simulink model "ABB_1010"  (R2024a)
settings: Solver=VariableStepAuto  StartTime=0.0  StopTime=200  RelTol=1e-3
model workspace: external: MATLAB File C:\Users\lucas\OneDrive\Documents\MATLAB\projeto final\ABB_1010_DataFile.m (data not in the file)
values from neighbouring files (symbols this model uses):
  g = 9.81    [inicializacaoAntropomorfico.m]
  I1 = [ 0.00243841  0.00000307  0.00007261    [inicializacaoAntropomorfico.m]
  I2 = [ 0.01633569  0.00000387 -0.00034405    [inicializacaoAntropomorfico.m]
  I3 = [ 0.00244760 -0.00000208  0.00000538    [inicializacaoAntropomorfico.m]
  I4 = [ 0.00245792 -0.00000008  0.00003121    [inicializacaoAntropomorfico.m]
  I5 = [ 0.00062165 -0.00000206 -0.00000303    [inicializacaoAntropomorfico.m]
  I6 = [ 0.00000357  0.00000000  0.00000000    [inicializacaoAntropomorfico.m]
  I7 = [(m7*L7^2)/12 0.00000000  0.00000000    [inicializacaoAntropomorfico.m]
  L = [L1, L2, L3, L4, L5, L6, L7]    [inicializacaoAntropomorfico.m]
  Lcm1 = [-0.00258308  0.00024508 -0.01434968]    [inicializacaoAntropomorfico.m]
  Lcm2 = [-0.02078894  0.00020016 -0.10516734]    [inicializacaoAntropomorfico.m]
  Lcm3 = [ 0.00021912  0.00015355 -0.06228290]    [inicializacaoAntropomorfico.m]
  Lcm4 = [-0.00172658 -0.00124140 -0.07369196]    [inicializacaoAntropomorfico.m]
  Lcm5 = [-0.00014110  0.00085992 -0.03825278]    [inicializacaoAntropomorfico.m]
  Lcm6 = [ 0.00002478  0.00000000 -0.00042157]    [inicializacaoAntropomorfico.m]
  Lcm7 = [ 0           0          -0.05000000]    [inicializacaoAntropomorfico.m]
  m = [m1, m2, m3, m4, m5, m6, m7]    [inicializacaoAntropomorfico.m]
  Pf = [  0.05    [inicializacaoAntropomorfico.m]
  Pi = [  0.2    [inicializacaoAntropomorfico.m]
  Raio = [0]    [inicializacaoAntropomorfico.m]
  Sentido = [0]    [inicializacaoAntropomorfico.m]
  Tipo = [1]    [inicializacaoAntropomorfico.m]
undefined symbols (not defined in the file or in its folder): smiData, X, Y, Z
libraries: sm_lib x35, nesl_utility x7
(part 2 of 16)

== matlab function ABB_1010/Dinamica1/MATLAB Function ==
  data: M output; I1 parameter; L parameter; Lcm1 parameter; Q input; I2 parameter; I3 parameter; I4 parameter; I5 parameter; I6 parameter; Lcm2 parameter; Lcm3 parameter; Lcm4 parameter; Lcm5 parameter; Lcm6 parameter; m parameter; Lcm7 parameter; I7 parameter
function M = func_M(I1, L, Lcm1, Q, I2, I3, I4, I5, I6, Lcm2, Lcm3, Lcm4, Lcm5, Lcm6, m, Lcm7, I7)
%func_M
%    OUT1 = func_M(Ixx2,Ixx3,Ixx4,Ixx5,Ixx6,Ixy2,Ixy3,Ixy4,Ixy5,Ixy6,Ixz2,Ixz3,Ixz4,Ixz5,Ixz6,Iyx2,Iyx3,Iyx4,Iyx5,Iyx6,Iyy2,Iyy3,Iyy4,Iyy5,Iyy6,Iyz2,Iyz3,Iyz4,Iyz5,Iyz6,Izx2,Izx3,Izx4,Izx5,Izx6,Izy2,Izy3,Izy4,Izy5,Izy6,Izz1,Izz2,Izz3,Izz4,Izz5,Izz6,Lx2,Lx3,Lxcm1,Lxcm2,Lxcm3,Lxcm4,Lxcm5,Lxcm6,Lycm1,Lycm2,Lycm3,Lycm4,Lycm5,Lycm6,Lz4,Lz5,Lzcm2,Lzcm3,Lzcm4,Lzcm5,Lzcm6,Q1,Q2,Q3,Q4,Q5,Q6,M1,M2,M3,M4,M5,M6)
    
%    This function was generated by the Symbolic Math Toolbox version 24.1.
%    30-Apr-2025 07:30:44

M = zeros(6,6);

m1  = m(1);
m2  = m(2);
m3  = m(3);
m4  = m(4);
m5  = m(5);
m6  = m(6);
m7  = m(7);

Q1  = Q(1);
Q2  = Q(2);
Q3  = Q(3);
Q4  = Q(4);
Q5  = Q(5);
Q6  = Q(6);

Lz1 = L(1);
Lx2 = L(2);
Lx3 = L(3);
Lx4 = L(4);
Lz5 = L(5);
Lz6 = L(6);
Lz7 = L(7);

Lxcm1 = Lcm1(1);
Lycm1 = Lcm1(2);
Lzcm1 = Lcm1(3);

Lxcm2 = Lcm2(1);
Lycm2 = Lcm2(2);
Lzcm2 = Lcm2(3);

Lxcm3 = Lcm3(1);
Lycm3 = Lcm3(2);
Lzcm3 = Lcm3(3);

Lxcm4 = Lcm4(1);
Lycm4 = Lcm4(2);
Lzcm4 = Lcm4(3);

Lxcm5 = Lcm5(1);
Lycm5 = Lcm5(2);
Lzcm5 = Lcm5(3);

Lxcm6 = Lcm6(1);
Lycm6 = Lcm6(2);
Lzcm6 = Lcm6(3);

Lxcm7 = Lcm7(1);
Lycm7 = Lcm7(2);
Lzcm7 = Lcm7(3);

Ixx1 = I1(1,1);
Ixy1 = I1(1,2);
Ixz1 = I1(1,3);
Iyx1 = I1(2,1);
Iyy1 = I1(2,2);
Iyz1 = I1(2,3);
Izx1 = I1(3,1);
Izy1 = I1(3,2);
Izz1 = I1(3,3);

Ixx2 = I2(1,1);
Ixy2 = I2(1,2);
Ixz2 = I2(1,3);
Iyx2 = I2(2,1);
Iyy2 = I2(2,2);
Iyz2 = I2(2,3);
Izx2 = I2(3,1);
Izy2 = I2(3,2);
Izz2 = I2(3,3);

Ixx3 = I3(1,1);
Ixy3 = I3(1,2);
Ixz3 = I3(1,3);
Iyx3 = I3(2,1);
Iyy3 = I3(2,2);
Iyz3 = I3(2,3);
Izx3 = I3(3,1);
Izy3 = I3(3,2);
Izz3 = I3(3,3);

Ixx4 = I4(1,1);
Ixy4 = I4(1,2);
Ixz4 = I4(1,3);
Iyx4 = I4(2,1);
Iyy4 = I4(2,2);
Iyz4 = I4(2,3);
Izx4 = I4(3,1);
Izy4 = I4(3,2);
Izz4 = I4(3,3);

Ixx5 = I5(1,1);
Ixy5 = I5(1,2);
Ixz5 = I5(1,3);
Iyx5 = I5(2,1);
Iyy5 = I5(2,2);
Iyz5 = I5(2,3);
Izx5 = I5(3,1);
Izy5 = I5(3,2);
Izz5 = I5(3,3);

Ixx6 = I6(1,1);
Ixy6 = I6(1,2);
Ixz6 = I6(1,3);
Iyx6 = I6(2,1);
Iyy6 = I6(2,2);
Iyz6 = I6(2,3);
Izx6 = I6(3,1);
Izy6 = I6(3,2);
Izz6 = I6(3,3);

Ixx7 = I7(1,1);
Ixy7 = I7(1,2);
Ixz7 = I7(1,3);
Iyx7 = I7(2,1);
Iyy7 = I7(2,2);
Iyz7 = I7(2,3);
Izx7 = I7(3,1);
Izy7 = I7(3,2);
Izz7 = I7(3,3);

t2 = cos(Q1);
t3 = cos(Q2);
t4 = cos(Q3);
t5 = cos(Q4);
t6 = cos(Q5);
t7 = cos(Q6);
t8 = sin(Q1);
t9 = sin(Q2);
t10 = sin(Q3);
t11 = sin(Q4);
t12 = sin(Q5);
t13 = sin(Q6);
t14 = Q2+Q3;
t15 = Lx2^2;
t16 = Lx3^2;
t17 = Lx4^2;
t18 = Lxcm3^2;
t19 = Lxcm4^2;
t20 = Lxcm5^2;
t21 = Lxcm6^2;
t22 = Lycm4^2;
t23 = Lycm5^2;
t24 = Lycm6^2;
t25 = Lz6^2;
t26 = Lzcm3^2;
t27 = Lzcm4^2;
t28 = Lzcm5^2;
t29 = Lzcm6^2;
t30 = Q4*2.0;
t31 = Q5*2.0;
t32 = Q6*2.0;
t33 = Lz6+Lzcm6;
t50 = Lx3*Lxcm3*m3*2.0;
t51 = Lz6*Lzcm6*m6*2.0;
t34 = t5^2;
t35 = t6^2;
t36 = t7^2;
t37 = sin(t30);
t38 = sin(t31);
t39 = sin(t32);
t40 = t11^2;
t41 = t12^2;
t42 = t13^2;
t43 = Ixx6*t5;
t44 = Iyy5*t5;
t45 = Izz6*t6;
t46 = Lycm6*t7;
t47 = cos(t14);
t48 = Lxcm6*t13;
t49 = sin(t14);
t52 = m3*t16;
t53 = m4*t16;
t54 = m5*t16;
t55 = m6*t16;
t56 = m3*t18;
t57 = m5*t20;
t58 = m6*t21;
t59 = m4*t22;
t60 = m5*t23;
t61 = m6*t24;
t62 = m6*t25;
t63 = m3*t26;
t64 = m4*t27;
t65 = m5*t28;
t66 = m6*t29;
t67 = t2*t5;
t68 = t2*t11;
t69 = t5*t8;
t70 = t8*t11;
t71 = Ixx5*t3*t4;
t72 = Iyy6*t3*t4;
t73 = Izz4*t3*t4;
t74 = Lx2*t2*t3;
t75 = Lx2*Lx3*m3*t4;
t76 = Lx2*Lx3*m4*t4;
t77 = Lx2*Lx3*m5*t4;
t78 = Lx2*Lx3*m6*t4;
t79 = Lx2*Lxcm3*m3*t4;
t80 = Lx3*Lxcm5*m5*t6;
t81 = Lx4*Lxcm6*m6*t7;
t82 = Lycm2*Lzcm2*m2*t3;
t83 = Lycm4*Lzcm4*m4*t5;
t84 = Lycm5*Lzcm5*m5*t6;
t85 = Lx2*t3*t8;
t86 = Lx2*Lycm2*m2*t9;
t87 = Lx2*Lycm3*m3*t9;
t88 = Lx4*Lycm6*m6*t13;
t89 = Lxcm2*Lycm2*m2*t9;
t90 = Lxcm5*Lycm5*m5*t12;
t91 = Lxcm6*Lycm6*m6*t12;
t92 = Lx3*Lz6*m6*t12;
t93 = Lx2*Lzcm3*m3*t10;
t94 = Lx2*Lzcm4*m4*t10;
t95 = Lx4*Lzcm4*m4*t11;
t96 = Lx3*Lzcm5*m5*t12;
t97 = Lx3*Lzcm6*m6*t12;
t98 = Lxcm4*Lzcm4*m4*t11;
t99 = Lxcm5*Lzcm5*m5*t11;
t100 = Ixx5*t9*t10;
t101 = Iyy6*t9*t10;
t102 = Izz4*t9*t10;
t103 = Izz6*t11*t12;
t118 = Lx3*Lx4*m4*t5*2.0;
t119 = Lx3*Lx4*m5*t5*2.0;
t120 = Lx3*Lx4*m6*t5*2.0;
t121 = Lx3*Lxcm4*m4*t5*2.0;
t122 = t5*t51;
t123 = Lx3*Lycm4*m4*t11*2.0;
t124 = Lx3*Lycm5*m5*t11*2.0;
t133 = t2*t3*t4;
t135 = t2*t3*t10;
t136 = t2*t4*t9;
t137 = t3*t4*t8;
t138 = t2*t9*t10;
t139 = t3*t8*t10;
t140 = t4*t8*t9;
t141 = t8*t9*t10;
t170 = Lx2*Lx4*m4*t3*t5;
t171 = Lx2*Lx4*m4*t4*t5;
t172 = Lx2*Lx4*m5*t3*t5;
t173 = Lx2*Lx4*m5*t4*t5;
t174 = Lx2*Lx4*m6*t3*t5;
t175 = Lx2*Lx4*m6*t4*t5;
t176 = Lx2*Lxcm4*m4*t3*t5;
t177 = Lx2*Lxcm4*m4*t4*t5;
t178 = Lx2*Lxcm5*m5*t4*t6;
t179 = Lx4*Lxcm5*m5*t5*t6;
t180 = Lx3*Lxcm6*m6*t6*t7;
t183 = Lycm3*Lzcm3*m3*t3*t4;
t189 = Lx3*Lycm3*m3*t3*t10;
t190 = Lx3*Lycm3*m3*t4*t9;
t191 = Lx2*Lycm4*m4*t3*t11;
t192 = Lx2*Lycm4*m4*t5*t9;
t193 = Lx2*Lycm4*m4*t4*t11;
t194 = Lx2*Lycm4*m4*t5*t10;
t195 = Lx4*Lycm4*m4*t3*t10;
t196 = Lx4*Lycm4*m4*t4*t9;
t197 = Lx2*Lycm5*m5*t3*t11;
t198 = Lx2*Lycm5*m5*t5*t9;
t199 = Lx2*Lycm5*m5*t4*t11;
t200 = Lx2*Lycm5*m5*t5*t10;
t201 = Lx4*Lycm5*m5*t3*t10;
t202 = Lx4*Lycm5*m5*t4*t9;
t203 = Lx3*Lycm6*m6*t6*t13;
t205 = Lxcm3*Lycm3*m3*t3*t10;
t206 = Lxcm3*Lycm3*m3*t4*t9;
t207 = Lxcm4*Lycm4*m4*t3*t10;
t208 = Lxcm4*Lycm4*m4*t4*t9;
t210 = Lxcm5*Lycm5*m5*t6*t11;
t212 = Lxcm6*Lycm6*m6*t6*t11;
t213 = Lx2*Lz6*m6*t4*t12;
t214 = Lx2*Lz6*m6*t6*t10;
t215 = Lx4*Lz6*m6*t5*t12;
t216 = Lx4*Lz6*m6*t6*t11;
t217 = Lx2*Lzcm5*m5*t4*t12;
t218 = Lx2*Lzcm5*m5*t6*t10;
t219 = Lx2*Lzcm6*m6*t4*t12;
t220 = Lx2*Lzcm6*m6*t6*t10;
t221 = Lx4*Lzcm5*m5*t5*t12;
t222 = Lx4*Lzcm5*m5*t6*t11;
t223 = Lx4*Lzcm6*m6*t5*t12;
t224 = Lx4*Lzcm6*m6*t6*t11;
t226 = Lxcm6*Lz6*m6*t7*t11;
t228 = Lxcm6*Lz6*m6*t7*t12;
t230 = Lxcm6*Lzcm6*m6*t7*t11;
t232 = Lxcm6*Lzcm6*m6*t7*t12;
t233 = Ixx6*t3*t10*t11;
t234 = Ixx6*t4*t9*t11;
t235 = Ixx5*t6*t11*t12;
t236 = Ixx6*t7*t12*t13;
t237 = Iyy5*t3*t10*t11;
t238 = Iyy5*t4*t9*t11;
t239 = Iyy6*t6*t11*t12;
t240 = Iyy6*t7*t12*t13;
t242 = Izz5*t6*t11*t12;
t244 = Lx2*Lx4*m4*t9*t11;
t245 = Lx2*Lx4*m4*t10*t11;
t246 = Lx2*Lx4*m5*t9*t11;
t247 = Lx2*Lx4*m5*t10*t11;
t248 = Lx2*Lx4*m6*t9*t11;
t249 = Lx2*Lx4*m6*t10*t11;
t250 = Lx2*Lxcm4*m4*t9*t11;
t251 = Lx2*Lxcm4*m4*t10*t11;
t252 = Lx2*Lxcm5*m5*t10*t12;
t253 = Lx4*Lxcm5*m5*t11*t12;
t255 = Lycm6*Lz6*m6*t11*t13;
t256 = Lycm6*Lz6*m6*t12*t13;
t257 = Lycm3*Lzcm3*m3*t9*t10;
t258 = Lycm5*Lzcm5*m5*t11*t12;
t259 = Lycm6*Lzcm6*m6*t11*t13;
t260 = Lycm6*Lzcm6*m6*t12*t13;
t261 = m4*t9*t10*t17;
t262 = m5*t9*t10*t17;
t263 = m6*t9*t10*t17;
t264 = m4*t9*t10*t19;
t298 = Lx4*Lxcm4*m4*t3*t4*2.0;
t300 = t3*t4*t51;
t305 = m4*t3*t4*t17;
t306 = m5*t3*t4*t17;
t307 = m6*t3*t4*t17;
t308 = m4*t3*t4*t19;
t315 = Lx4*Lxcm4*m4*t9*t10*2.0;
t317 = t9*t10*t51;
t331 = Lx3*Lx4*m4*t3*t4*t5;
t332 = Lx3*Lx4*m5*t3*t4*t5;
t333 = Lx3*Lx4*m6*t3*t4*t5;
t334 = Lx3*Lxcm4*m4*t3*t4*t5;
t335 = Lx2*Lxcm5*m5*t3*t5*t6;
t337 = Lx2*Lxcm6*m6*t3*t5*t7;
t339 = Lx2*Lxcm6*m6*t4*t6*t7;
t350 = Lx3*Lycm4*m4*t3*t4*t11;
t351 = Lx3*Lycm4*m4*t3*t5*t10;
t352 = Lx3*Lycm4*m4*t4*t5*t9;
t353 = Lx3*Lycm5*m5*t3*t4*t11;
t354 = Lx3*Lycm5*m5*t3*t5*t10;
t355 = Lx3*Lycm5*m5*t4*t5*t9;
t356 = Lx2*Lycm6*m6*t3*t5*t13;
t364 = Lx2*Lycm6*m6*t4*t6*t13;
t369 = Lxcm5*Lycm5*m5*t3*t6*t10;
t370 = Lxcm5*Lycm5*m5*t4*t6*t9;
t372 = Lxcm6*Lycm6*m6*t3*t6*t10;
t373 = Lxcm6*Lycm6*m6*t4*t6*t9;
t374 = Lx2*Lz6*m6*t3*t5*t12;
t375 = Lx2*Lz6*m6*t3*t6*t11;
t379 = Lx4*Lzcm4*m4*t3*t5*t10;
t380 = Lx4*Lzcm4*m4*t4*t5*t9;
t381 = Lx2*Lzcm5*m5*t3*t5*t12;
t382 = Lx2*Lzcm5*m5*t3*t6*t11;
t385 = Lx2*Lzcm6*m6*t3*t5*t12;
t386 = Lx2*Lzcm6*m6*t3*t6*t11;
t392 = Lxcm4*Lzcm4*m4*t3*t5*t10;
t393 = Lxcm4*Lzcm4*m4*t4*t5*t9;
t395 = Lxcm5*Lzcm5*m5*t3*t5*t10;
t396 = Lxcm5*Lzcm5*m5*t4*t5*t9;
t402 = Ixx4*t3*t5*t10*t11;
t403 = Ixx4*t4*t5*t9*t11;
t407 = Ixx6*t6*t7*t11*t13;
t408 = Iyy4*t3*t5*t10*t11;
t409 = Iyy4*t4*t5*t9*t11;
t413 = Iyy6*t6*t7*t11*t13;
t414 = Izz5*t3*t5*t10*t11;
t415 = Izz5*t4*t5*t9*t11;
t416 = Izz6*t3*t5*t10*t11;
t417 = Izz6*t4*t5*t9*t11;
t418 = Izz6*t3*t5*t10*t12;
t419 = Izz6*t4*t5*t9*t12;
t422 = Lx3*Lx4*m4*t3*t10*t11;
t423 = Lx3*Lx4*m4*t4*t9*t11;
t424 = Lx3*Lx4*m4*t5*t9*t10;
t425 = Lx3*Lx4*m5*t3*t10*t11;
t426 = Lx3*Lx4*m5*t4*t9*t11;
t427 = Lx3*Lx4*m5*t5*t9*t10;
t428 = Lx3*Lx4*m6*t3*t10*t11;
t429 = Lx3*Lx4*m6*t4*t9*t11;
t430 = Lx3*Lx4*m6*t5*t9*t10;
t431 = Lx3*Lxcm4*m4*t3*t10*t11;
t432 = Lx3*Lxcm4*m4*t4*t9*t11;
t433 = Lx3*Lxcm4*m4*t5*t9*t10;
t434 = Lx2*Lxcm5*m5*t3*t11*t12;
t435 = Lx2*Lxcm5*m5*t6*t9*t11;
t437 = Lx2*Lxcm5*m5*t6*t10*t11;
t442 = Lx2*Lxcm6*m6*t7*t10*t11;
t447 = Lx2*Lxcm6*m6*t7*t10*t12;
t452 = Lycm4*Lzcm4*m4*t3*t10*t11;
t453 = Lycm4*Lzcm4*m4*t4*t9*t11;
t455 = Lycm5*Lzcm5*m5*t3*t10*t12;
t456 = Lycm5*Lzcm5*m5*t4*t9*t12;
t460 = Lx3*Lycm4*m4*t9*t10*t11;
t461 = Lx3*Lycm5*m5*t9*t10*t11;
t462 = Lx2*Lycm6*m6*t10*t11*t13;
t464 = Lx2*Lycm6*m6*t10*t12*t13;
t468 = Lx2*Lz6*m6*t9*t11*t12;
t469 = Lx2*Lz6*m6*t10*t11*t12;
t471 = Lx2*Lzcm5*m5*t9*t11*t12;
t472 = Lx2*Lzcm5*m5*t10*t11*t12;
t473 = Lx2*Lzcm6*m6*t9*t11*t12;
t474 = Lx2*Lzcm6*m6*t10*t11*t12;
t535 = Lz6*Lzcm6*m6*t9*t10*-2.0;
t555 = Lx4*Lxcm5*m5*t3*t4*t6*2.0;
t567 = Lx4*Lz6*m6*t3*t4*t12*2.0;
t568 = Lx4*Lzcm5*m5*t3*t4*t12*2.0;
t569 = Lx4*Lzcm6*m6*t3*t4*t12*2.0;
t574 = Lx4*Lxcm5*m5*t6*t9*t10*2.0;
t579 = t3*t10*t11*t51;
t580 = t4*t9*t11*t51;
t582 = Lx4*Lz6*m6*t9*t10*t12*2.0;
t583 = Lx4*Lzcm5*m5*t9*t10*t12*2.0;
t584 = Lx4*Lzcm6*m6*t9*t10*t12*2.0;
t613 = Lx3*Lxcm6*m6*t3*t4*t5*t7;
t628 = Lx3*Lycm6*m6*t3*t4*t5*t13;
t643 = Lx3*Lz6*m6*t3*t4*t6*t11;
t645 = Lx4*Lz6*m6*t3*t5*t6*t10;
t646 = Lx4*Lz6*m6*t4*t5*t6*t9;
t648 = Lx3*Lzcm5*m5*t3*t4*t6*t11;
t650 = Lx4*Lzcm5*m5*t3*t5*t6*t10;
t651 = Lx4*Lzcm5*m5*t4*t5*t6*t9;
t653 = Lx3*Lzcm6*m6*t3*t4*t6*t11;
t655 = Lx4*Lzcm6*m6*t3*t5*t6*t10;
t656 = Lx4*Lzcm6*m6*t4*t5*t6*t9;
t658 = Lxcm6*Lz6*m6*t3*t5*t7*t10;
t659 = Lxcm6*Lz6*m6*t4*t5*t7*t9;
t663 = Lxcm6*Lzcm6*m6*t3*t5*t7*t10;
t664 = Lxcm6*Lzcm6*m6*t4*t5*t7*t9;
t671 = Ixx5*t3*t5*t6*t10*t12;
t672 = Ixx5*t4*t5*t6*t9*t12;
t674 = Ixx6*t3*t6*t7*t10*t13;
t675 = Ixx6*t4*t6*t7*t9*t13;
t677 = Iyy6*t3*t5*t6*t10*t12;
t678 = Iyy6*t4*t5*t6*t9*t12;
t680 = Iyy6*t3*t6*t7*t10*t13;
t681 = Iyy6*t4*t6*t7*t9*t13;
t683 = Izz5*t3*t5*t6*t10*t12;
t684 = Izz5*t4*t5*t6*t9*t12;
t691 = Lx3*Lxcm5*m5*t3*t4*t11*t12;
t696 = Lx4*Lxcm5*m5*t3*t5*t10*t12;
t697 = Lx4*Lxcm5*m5*t3*t6*t10*t11;
t698 = Lx4*Lxcm5*m5*t4*t5*t9*t12;
t699 = Lx4*Lxcm5*m5*t4*t6*t9*t11;
t703 = Lx3*Lxcm6*m6*t5*t7*t9*t10;
t705 = Lx2*Lxcm6*m6*t3*t7*t11*t12;
t706 = Lx2*Lxcm6*m6*t6*t7*t9*t11;
t711 = Lycm6*Lz6*m6*t3*t5*t10*t13;
t713 = Lycm6*Lz6*m6*t4*t5*t9*t13;
t725 = Lycm6*Lzcm6*m6*t3*t5*t10*t13;
t727 = Lycm6*Lzcm6*m6*t4*t5*t9*t13;
t736 = Lx3*Lycm6*m6*t5*t9*t10*t13;
t738 = Lx2*Lycm6*m6*t3*t11*t12*t13;
t739 = Lx2*Lycm6*m6*t6*t9*t11*t13;
t751 = Lx3*Lz6*m6*t6*t9*t10*t11;
t752 = Lx4*Lz6*m6*t3*t10*t11*t12;
t753 = Lx4*Lz6*m6*t4*t9*t11*t12;
t758 = Lx3*Lzcm5*m5*t6*t9*t10*t11;
t759 = Lx4*Lzcm5*m5*t3*t10*t11*t12;
t760 = Lx4*Lzcm5*m5*t4*t9*t11*t12;
t765 = Lx3*Lzcm6*m6*t6*t9*t10*t11;
t766 = Lx4*Lzcm6*m6*t3*t10*t11*t12;
t767 = Lx4*Lzcm6*m6*t4*t9*t11*t12;
t789 = Lx3*Lxcm5*m5*t9*t10*t11*t12;
t867 = Lz6*Lzcm6*m6*t6*t11*t12*-2.0;
t909 = Lxcm5*Lzcm5*m5*t3*t4*t6*t12*2.0;
t912 = Lx4*Lxcm4*m4*t3*t5*t10*t11*2.0;
t913 = Lx4*Lxcm4*m4*t4*t5*t9*t11*2.0;
t925 = Lxcm5*Lzcm5*m5*t6*t9*t10*t12*2.0;
t927 = m4*t3*t5*t10*t11*t17;
t928 = m4*t4*t5*t9*t11*t17;
t929 = m5*t3*t5*t10*t11*t17;
t930 = m5*t4*t5*t9*t11*t17;
t931 = m6*t3*t5*t10*t11*t17;
t932 = m6*t4*t5*t9*t11*t17;
t933 = m4*t3*t5*t10*t11*t19;
t934 = m4*t4*t5*t9*t11*t19;
t1007 = Lx3*Lxcm6*m6*t3*t4*t7*t11*t12;
t1032 = Lx3*Lycm6*m6*t3*t4*t11*t12*t13;
t1061 = Lx3*Lxcm6*m6*t7*t9*t10*t11*t12;
t1071 = Lx3*Lycm6*m6*t9*t10*t11*t12*t13;
t104 = Ixx4*t34;
t105 = Ixx5*t35;
t106 = Ixx6*t34;
t107 = Ixx6*t36;
t108 = Iyy4*t34;
t109 = Iyy5*t34;
t110 = Iyy6*t35;
t111 = Iyy6*t36;
t112 = Izz5*t34;
t113 = Izz5*t35;
t114 = Izz6*t34;
t115 = Izz6*t35;
t116 = t47^2;
t117 = t49^2;
t125 = t5*t57;
t126 = t6*t58;
t127 = t5*t61;
t128 = t6*t61;
t129 = t5*t62;
t130 = t5*t65;
t131 = t5*t66;
t132 = t6*t47;
t134 = t12*t47;
t144 = -t82;
t145 = -t83;
t146 = -t84;
t147 = -t123;
t148 = -t124;
t149 = -t88;
t150 = -t91;
t151 = -t95;
t152 = -t98;
t153 = -t100;
t154 = -t101;
t155 = -t102;
t156 = t36*t43;
t158 = Lx4*Lycm4*m4*t37;
t159 = Lx4*Lycm5*m5*t37;
t160 = Lxcm4*Lycm4*m4*t37;
t161 = Lxcm6*Lycm6*m6*t39;
t162 = Lxcm5*Lzcm5*m5*t38;
t168 = t3*t4*t45;
t169 = Lycm3*Lzcm3*m3*t47;
t181 = Lz6*m6*t5*t46;
t182 = Lz6*m6*t6*t46;
t184 = t5*t84;
t185 = Lzcm6*m6*t5*t46;
t186 = Lzcm6*m6*t6*t46;
t187 = Lx3*Lycm3*m3*t49;
t188 = Lxcm3*Lycm3*m3*t49;
t204 = Lx3*m6*t12*t46;
t209 = t5*t90;
t211 = t5*t91;
t225 = Lz6*m6*t5*t48;
t227 = Lz6*m6*t6*t48;
t229 = Lzcm6*m6*t5*t48;
t231 = Lzcm6*m6*t6*t48;
t241 = t9*t10*t45;
t243 = t11*t12*t45;
t254 = Lx3*m6*t12*t48;
t265 = t9*t10*t58;
t266 = t11*t12*t58;
t267 = t9*t10*t59;
t268 = t9*t10*t60;
t269 = t11*t12*t61;
t270 = t9*t10*t62;
t271 = t9*t10*t65;
t272 = t9*t10*t66;
t273 = t46+t48;
t274 = t5*t6*t49;
t275 = t5*t12*t49;
t276 = Lx4*Lxcm4*m4*t34*2.0;
t277 = t34*t51;
t278 = t35*t51;
t279 = m4*t17*t34;
t280 = m5*t17*t34;
t281 = m6*t17*t34;
t282 = m4*t19*t34;
t283 = t35*t57;
t284 = t34*t58;
t285 = t36*t58;
t286 = t34*t59;
t287 = t34*t60;
t288 = t35*t61;
t289 = t36*t61;
t290 = t34*t62;
t291 = t35*t62;
t292 = t34*t65;
t293 = t35*t65;
t294 = t34*t66;
t295 = t35*t66;
t296 = -t138;
t297 = -t141;
t299 = t5*t80*2.0;
t301 = Lx3*m6*t11*t46*2.0;
t302 = t5*t92*2.0;
t303 = t5*t96*2.0;
t304 = t5*t97*2.0;
t309 = t3*t4*t58;
t310 = t3*t4*t59;
t311 = t3*t4*t60;
t312 = t3*t4*t62;
t313 = t3*t4*t65;
t314 = t3*t4*t66;
t316 = Lx3*m6*t11*t48*2.0;
t318 = t35*t71;
t320 = t35*t72;
t321 = t36*t72;
t324 = t35*t100;
t326 = t35*t101;
t327 = t36*t101;
t336 = t5*t178;
t338 = t3*t4*t81;
t340 = t5*t6*t81;
t349 = Lx3*Lycm5*m5*t5*t49;
t357 = Lx2*m6*t3*t11*t46;
t358 = Lx2*m6*t5*t9*t46;
t359 = Lx2*m6*t4*t11*t46;
t360 = Lx2*m6*t5*t10*t46;
t361 = t3*t4*t88;
t362 = Lx4*m6*t3*t10*t46;
t363 = Lx4*m6*t4*t9*t46;
t365 = Lx2*m6*t4*t12*t46;
t366 = t5*t6*t88;
t367 = Lx4*m6*t5*t12*t46;
t368 = t3*t4*t90;
t371 = t3*t4*t91;
t376 = t5*t213;
t377 = t5*t214;
t383 = t5*t217;
t384 = t5*t218;
t387 = t5*t219;
t388 = t5*t220;
t390 = t6*t226;
t394 = t3*t4*t99;
t398 = t6*t230;
t399 = Ixx4*t5*t11*t49;
t400 = Iyy4*t5*t11*t49;
t401 = t11*t44*t49;
t404 = t3*t10*t11*t43;
t405 = t4*t9*t11*t43;
t406 = t7*t12*t13*t43;
t410 = t3*t10*t11*t44;
t411 = t4*t9*t11*t44;
t412 = t5*t240;
out1 = ft_1({Ixx2,Ixx3,Ixx4,Ixx5,Ixx6,Iyy2,Iyy3,Iyy4,Iyy5,Iyy6,Izz1,Izz2,Izz3,Izz4,Izz5,Izz6,Lx2,Lx3,Lx4,Lxcm1,Lxcm2,Lxcm3,Lxcm4,Lxcm5,Lxcm6,Lycm1,Lycm2,Lycm3,Lycm4,Lycm5,Lycm6,Lz6,Lzcm2,Lzcm3,Lzcm4,Lzcm5,Lzcm6,m1,m2,m3,m4,m5,m6,t10,t100,t1007,t101,t103,t1032,t104,t105,t106,t1061,t107,t1071,t108,t109,t11,t110,t111,t112,t113,t114,t115,t116,t117,t118,t119,t12,t120,t121,t122,t125,t126,t127,t128,t129,t13,t130,t131,t132,t133,t134,t135,t136,t137,t139,t140,t144,t145,t146,t147,t148,t149,t15,t150,t151,t152,t153,t154,t155,t156,t158,t159,t160,t161,t162,t168,t169,t17,t170,t171,t172,t173,t174,t175,t176,t177,t178,t179,t180,t181,t182,t183,t184,t185,t186,t187,t188,t189,t19,t190,t191,t192,t193,t194,t195,t196,t197,t198,t199,t2,t200,t201,t202,t203,t204,t205,t206,t207,t208,t209,t210,t211,t212,t213,t214,t215,t216,t217,t218,t219,t220,t221,t222,t223,t224,t225,t226,t227,t228,t229,t230,t231,t232,t233,t234,t235,t236,t237,t238,t239,t240,t241,t242,t243,t244,t245,t246,t247,t248,t249,t250,t251,t252,t253,t254,t255,t256,t257,t258,t259,t260,t261,t262,t263,t264,t265,t266,t267,t268,t269,t270,t271,t272,t273,t274,t275,t276,t277,t278,t279,t280,t281,t282,t283,t284,t285,t286,t287,t288,t289,t290,t291,t292,t293,t294,t295,t296,t297,t298,t299,t3,t300,t301,t302,t303,t304,t305,t306,t307,t308,t309,t310,t311,t312,t313,t314,t315,t316,t317,t318,t320,t321,t324,t326,t327,t33,t331,t332,t333,t334,t335,t336,t337,t338,t339,t34,t340,t349,t35,t350,t351,t352,t353,t354,t355,t356,t357,t358,t359,t36,t360,t361,t362,t363,t364,t365,t366,t367,t368,t369,t370,t371,t372,t373,t374,t375,t376,t377,t379,t380,t381,t382,t383,t384,t385,t386,t387,t388,t390,t392,t393,t394,t395,t396,t398,t399,t4,t40,t400,t401,t402,t403,t404,t405,t406,t407,t408,t409,t41,t410,t411,t412,t413,t414,t415,t416,t417,t418,t419,t42,t422,t423,t424,t425,t426,t427,t428,t429,t43,t430,t431,t432,t433,t434,t435,t437,t44,t442,t447,t45,t452,t453,t455,t456,t46,t460,t461,t462,t464,t468,t469,t47,t471,t472,t473,t474,t48,t49,t5,t50,t51,t52,t53,t535,t54,t55,t555,t56,t567,t568,t569,t57,t574,t579,t58,t580,t582,t583,t584,t59,t6,t60,t61,t613,t62,t628,t63,t64,t643,t645,t646,t648,t65,t650,t651,t653,t655,t656,t658,t659,t66,t663,t664,t67,t671,t672,t674,t675,t677,t678,t68,t680,t681,t683,t684,t69,t691,t696,t697,t698,t699,t7,t70,t703,t705,t706,t71,t711,t713,t72,t725,t727,t73,t736,t738,t739,t74,t75,t751,t752,t753,t758,t759,t76,t760,t765,t766,t767,t77,t78,t789,t79,t8,t80,t81,t83,t84,t85,t86,t867,t87,t88,t89,t9,t90,t909,t91,t912,t913,t92,t925,t927,t928,t929,t93,t930,t931,t932,t933,t934,t94,t95,t96,t97,t98,t99});
end
function out1 = ft_1(ct)
[Ixx2,Ixx3,Ixx4,Ixx5,Ixx6,Iyy2,Iyy3,Iyy4,Iyy5,Iyy6,Izz1,Izz2,Izz3,Izz4,Izz5,Izz6,Lx2,Lx3,Lx4,Lxcm1,Lxcm2,Lxcm3,Lxcm4,Lxcm5,Lxcm6,Lycm1,Lycm2,Lycm3,Lycm4,Lycm5,Lycm6,Lz6,Lzcm2,Lzcm3,Lzcm4,Lzcm5,Lzcm6,m1,m2,m3,m4,m5,m6,t10,t100,t1007,t101,t103,t1032,t104,t105,t106,t1061,t107,t1071,t108,t109,t11,t110,t111,t112,t113,t114,t115,t116,t117,t118,t119,t12,t120,t121,t122,t125,t126,t127,t128,t129,t13,t130,t131,t132,t133,t134,t135,t136,t137,t139,t140,t144,t145,t146,t147,t148,t149,t15,t150,t151,t152,t153,t154,t155,t156,t158,t159,t160,t161,t162,t168,t169,t17,t170,t171,t172,t173,t174,t175,t176,t177,t178,t179,t180,t181,t182,t183,t184,t185,t186,t187,t188,t189,t19,t190,t191,t192,t193,t194,t195,t196,t197,t198,t199,t2,t200,t201,t202,t203,t204,t205,t206,t207,t208,t209,t210,t211,t212,t213,t214,t215,t216,t217,t218,t219,t220,t221,t222,t223,t224,t225,t226,t227,t228,t229,t230,t231,t232,t233,t234,t235,t236,t237,t238,t239,t240,t241,t242,t243,t244,t245,t246,t247,t248,t249,t250,t251,t252,t253,t254,t255,t256,t257,t258,t259,t260,t261,t262,t263,t264,t265,t266,t267,t268,t269,t270,t271,t272,t273,t274,t275,t276,t277,t278,t279,t280,t281,t282,t283,t284,t285,t286,t287,t288,t289,t290,t291,t292,t293,t294,t295,t296,t297,t298,t299,t3,t300,t301,t302,t303,t304,t305,t306,t307,t308,t309,t310,t311,t312,t313,t314,t315,t316,t317,t318,t320,t321,t324,t326,t327,t33,t331,t332,t333,t334,t335,t336,t337,t338,t339,t34,t340,t349,t35,t350,t351,t352,t353,t354,t355,t356,t357,t358,t359,t36,t360,t361,t362,t363,t364,t365,t366,t367,t368,t369,t370,t371,t372,t373,t374,t375,t376,t377,t379,t380,t381,t382,t383,t384,t385,t386,t387,t388,t390,t392,t393,t394,t395,t396,t398,t399,t4,t40,t400,t401,t402,t403,t404,t405,t406,t407,t408,t409,t41,t410,t411,t412,t413,t414,t415,t416,t417,t418,t419,t42,t422,t423,t424,t425,t426,t427,t428,t429,t43,t430,t431,t432,t433,t434,t435,t437,t44,t442,t447,t45,t452,t453,t455,t456,t46,t460,t461,t462,t464,t468,t469,t47,t471,t472,t473,t474,t48,t49,t5,t50,t51,t52,t53,t535,t54,t55,t555,t56,t567,t568,t569,t57,t574,t579,t58,t580,t582,t583,t584,t59,t6,t60,t61,t613,t62,t628,t63,t64,t643,t645,t646,t648,t65,t650,t651,t653,t655,t656,t658,t659,t66,t663,t664,t67,t671,t672,t674,t675,t677,t678,t68,t680,t681,t683,t684,t69,t691,t696,t697,t698,t699,t7,t70,t703,t705,t706,t71,t711,t713,t72,t725,t727,t73,t736,t738,t739,t74,t75,t751,t752,t753,t758,t759,t76,t760,t765,t766,t767,t77,t78,t789,t79,t8,t80,t81,t83,t84,t85,t86,t867,t87,t88,t89,t9,t90,t909,t91,t912,t913,t92,t925,t927,t928,t929,t93,t930,t931,t932,t933,t934,t94,t95,t96,t97,t98,t99] = ct{:};
t420 = Lx3*Lx4*m5*t11*t49;
t421 = Lx3*Lx4*m6*t11*t49;
t436 = t5*t252;
t438 = Lx2*m6*t3*t11*t48;
t439 = Lx2*m6*t5*t9*t48;
t440 = Lx2*m6*t4*t11*t48;
t441 = Lx2*m6*t5*t10*t48;
t443 = Lx4*m6*t3*t10*t48;
t444 = Lx4*m6*t4*t9*t48;
t445 = t9*t10*t81;
t446 = Lx2*m6*t4*t12*t48;
t448 = Lx4*m6*t5*t12*t48;
t449 = t11*t12*t81;
t450 = t6*t255;
t451 = Lz6*m6*t11*t12*t46;
t454 = t9*t10*t83;
t457 = t9*t10*t84;
t458 = t6*t259;
t459 = Lzcm6*m6*t11*t12*t46;
t463 = t9*t10*t88;
t466 = t9*t10*t90;
t467 = t9*t10*t91;
t470 = t9*t10*t95;
t475 = Lz6*m6*t11*t12*t48;
t476 = t9*t10*t98;
t477 = t9*t10*t99;
t478 = Lzcm6*m6*t11*t12*t48;
t482 = -t183;
t494 = -t191;
t495 = -t193;
t496 = -t194;
t497 = -t195;
t498 = -t196;
t499 = -t197;
t500 = -t199;
t501 = -t200;
t502 = -t201;
t503 = -t202;
t504 = -t203;
t507 = -t207;
t508 = -t208;
t509 = -t210;
t511 = -t216;
t512 = -t222;
t513 = -t224;
t518 = -t235;
t519 = -t236;
t520 = -t239;
t522 = -t245;
t523 = -t247;
t524 = -t249;
t525 = -t251;
t526 = -t315;
t527 = -t252;
t530 = -t255;
t531 = -t256;
t532 = -t258;
t533 = -t259;
t534 = -t260;
t536 = -t261;
t537 = -t262;
t538 = -t263;
t539 = -t264;
t546 = Lx4*Lxcm5*m5*t6*t34*2.0;
t547 = t36*t91*2.0;
t548 = Lx4*Lz6*m6*t12*t34*2.0;
t549 = Lx4*Lzcm5*m5*t12*t34*2.0;
t550 = Lx4*Lzcm6*m6*t12*t34*2.0;
t551 = t35*t99*2.0;
t556 = t5*t180*2.0;
t562 = t5*t203*2.0;
t563 = Lx4*m6*t5*t11*t46*2.0;
t564 = t5*t210*2.0;
t565 = t5*t212*2.0;
t566 = m6*t5*t46*t48*2.0;
t570 = t6*t228*2.0;
t571 = t6*t232*2.0;
t575 = Lx4*m6*t5*t11*t48*2.0;
t576 = t6*t256*2.0;
t577 = t5*t258*2.0;
t578 = t6*t260*2.0;
t585 = t3*t10*t11*t57;
t586 = t4*t9*t11*t57;
t588 = t6*t11*t12*t57;
t589 = t7*t12*t13*t58;
t590 = t3*t10*t11*t61;
t591 = t4*t9*t11*t61;
t594 = t7*t12*t13*t61;
t595 = t3*t10*t11*t62;
t596 = t4*t9*t11*t62;
t597 = t6*t11*t12*t62;
t598 = t3*t10*t11*t65;
t599 = t4*t9*t11*t65;
t600 = t3*t10*t11*t66;
t601 = t4*t9*t11*t66;
t602 = t6*t11*t12*t65;
t603 = t6*t11*t12*t66;
t612 = t3*t4*t5*t80;
t614 = t6*t337;
t615 = t5*t339;
t620 = Lx3*m6*t5*t46*t49;
t629 = Lx3*m6*t3*t4*t11*t46;
t630 = Lx3*m6*t3*t5*t10*t46;
t631 = Lx3*m6*t4*t5*t9*t46;
t632 = t6*t356;
t634 = t5*t364;
t637 = t5*t369;
t638 = t5*t370;
t640 = t5*t372;
t641 = t5*t373;
t642 = t3*t4*t5*t92;
t647 = t3*t4*t5*t96;
t652 = t3*t4*t5*t97;
t657 = t3*t4*t226;
t661 = t3*t4*t228;
t662 = t3*t4*t230;
t666 = t3*t4*t232;
t670 = t6*t11*t12*t71;
t676 = t6*t11*t12*t72;
t679 = t7*t12*t13*t72;
t682 = t3*t4*t242;
t686 = t3*t5*t10*t12*t45;
t687 = t4*t5*t9*t12*t45;
t688 = t11*t49*t80;
t690 = Lx3*m6*t5*t48*t49;
t692 = t3*t10*t11*t80;
t693 = t4*t9*t11*t80;
t694 = t5*t9*t10*t80;
t695 = t3*t4*t253;
t700 = Lx3*m6*t3*t4*t11*t48;
t701 = Lx3*m6*t3*t5*t10*t48;
t702 = Lx3*m6*t4*t5*t9*t48;
t708 = t5*t447;
t709 = t6*t442;
t710 = t3*t4*t255;
t712 = Lz6*m6*t3*t10*t11*t46;
t714 = Lz6*m6*t4*t9*t11*t46;
t715 = t3*t4*t256;
t716 = Lz6*m6*t3*t10*t12*t46;
t717 = Lz6*m6*t4*t9*t12*t46;
t719 = t5*t455;
t721 = t5*t456;
t724 = t3*t4*t259;
t726 = Lzcm6*m6*t3*t10*t11*t46;
t728 = Lzcm6*m6*t4*t9*t11*t46;
t729 = t3*t4*t260;
t730 = Lzcm6*m6*t3*t10*t12*t46;
t731 = Lzcm6*m6*t4*t9*t12*t46;
t733 = t11*t49*t92;
t734 = t11*t49*t96;
t735 = t11*t49*t97;
t737 = Lx3*m6*t9*t10*t11*t46;
t740 = t5*t464;
t741 = t6*t462;
t742 = t3*t10*t11*t90;
t743 = t4*t9*t11*t90;
t748 = t3*t10*t11*t92;
t749 = t4*t9*t11*t92;
t750 = t5*t9*t10*t92;
t754 = t9*t10*t216;
t755 = t3*t10*t11*t96;
t756 = t4*t9*t11*t96;
t757 = t5*t9*t10*t96;
t761 = t9*t10*t222;
t762 = t3*t10*t11*t97;
t763 = t4*t9*t11*t97;
t764 = t5*t9*t10*t97;
t768 = t9*t10*t224;
t769 = Lz6*m6*t3*t10*t11*t48;
t770 = Lz6*m6*t4*t9*t11*t48;
t771 = t9*t10*t226;
t772 = Lz6*m6*t3*t10*t12*t48;
t773 = Lz6*m6*t4*t9*t12*t48;
t775 = t9*t10*t228;
t776 = Lzcm6*m6*t3*t10*t11*t48;
t777 = Lzcm6*m6*t4*t9*t11*t48;
t778 = t9*t10*t230;
t779 = Lzcm6*m6*t3*t10*t12*t48;
t780 = Lzcm6*m6*t4*t9*t12*t48;
t782 = t9*t10*t232;
t783 = t6*t11*t12*t100;
t784 = t9*t10*t236;
t785 = t6*t11*t12*t101;
t787 = t9*t10*t242;
t790 = t9*t10*t253;
t791 = Lx3*m6*t9*t10*t11*t48;
t792 = t9*t10*t255;
t793 = t9*t10*t256;
t794 = t9*t10*t259;
t795 = t9*t10*t260;
t800 = -t350;
t801 = -t353;
t802 = -t356;
t809 = -t364;
t815 = -t369;
t816 = -t370;
t825 = -t395;
t826 = -t396;
t831 = -t402;
t832 = -t403;
t834 = -t413;
t835 = -t414;
t836 = -t415;
t837 = -t416;
t838 = -t417;
t839 = -t418;
t840 = -t419;
t841 = -t424;
t842 = -t427;
t843 = -t430;
t844 = -t433;
t845 = -t434;
t847 = -t437;
t848 = -t574;
t852 = -t442;
t857 = -t447;
t861 = -t452;
t862 = -t453;
t863 = -t455;
t864 = -t456;
t870 = -t469;
t871 = -t582;
t872 = -t472;
t873 = -t583;
t874 = -t474;
t875 = -t584;
t883 = Lx4*Lycm5*m5*t34*t49;
t884 = t34*t195;
t885 = t34*t196;
t886 = t34*t207;
t887 = t34*t208;
t894 = Lx4*Lycm5*m5*t40*t49;
t895 = t35*t255*2.0;
t896 = t35*t259*2.0;
t908 = m6*t3*t4*t46*t48*2.0;
t910 = t6*t7*t11*t13*t43*2.0;
t911 = t5*t413*2.0;
t917 = t3*t10*t11*t122;
t918 = t4*t9*t11*t122;
t919 = m5*t5*t11*t17*t49;
t920 = m6*t5*t11*t17*t49;
t921 = t5*t11*t49*t60;
t923 = m6*t9*t10*t46*t48*2.0;
t935 = t3*t5*t10*t11*t58;
t936 = t4*t5*t9*t11*t58;
t937 = t3*t5*t10*t12*t58;
t938 = t4*t5*t9*t12*t58;
t941 = t3*t5*t10*t11*t59;
t942 = t4*t5*t9*t11*t59;
t943 = t3*t5*t10*t11*t60;
t944 = t4*t5*t9*t11*t60;
t971 = t6*t34*t81*2.0;
t975 = t34*t201*2.0;
t976 = t34*t202*2.0;
t977 = t6*t34*t88*2.0;
t981 = t36*t212*2.0;
t982 = m6*t34*t46*t48*2.0;
t983 = m6*t35*t46*t48*2.0;
t984 = t35*t226*2.0;
t985 = Lxcm5*Lzcm5*m5*t6*t12*t34*2.0;
t986 = t35*t230*2.0;
t999 = t3*t6*t7*t10*t13*t43;
t1000 = t4*t6*t7*t9*t13*t43;
t1002 = t5*t680;
t1003 = t5*t681;
t1004 = t11*t49*t180;
t1008 = t3*t10*t11*t180;
t1009 = t4*t9*t11*t180;
t1010 = t5*t9*t10*t180;
t1012 = t3*t5*t10*t12*t81;
t1013 = t3*t6*t10*t11*t81;
t1014 = t4*t5*t9*t12*t81;
t1015 = t4*t6*t9*t11*t81;
t1016 = t6*t711;
t1019 = t6*t713;
t1023 = t6*t725;
t1026 = t6*t727;
t1035 = t5*t9*t10*t203;
t1038 = t3*t5*t10*t12*t88;
t1041 = t4*t5*t9*t12*t88;
t1054 = t7*t12*t13*t233;
t1055 = t7*t12*t13*t234;
t1057 = t3*t10*t11*t240;
t1058 = t4*t9*t11*t240;
t1076 = -t628;
t1089 = -t658;
t1090 = -t659;
t1092 = -t663;
t1093 = -t664;
t1099 = -t680;
t1100 = -t681;
t1102 = -t683;
t1103 = -t684;
t1106 = -t691;
t1108 = -t696;
t1109 = -t698;
t1111 = -t703;
t1113 = -t705;
t1136 = -t739;
t1142 = -t751;
t1144 = -t758;
t1146 = -t765;
t1154 = -t925;
t1166 = Lz6*Lzcm6*m6*t34*t35*-2.0;
t1167 = Lx4*m6*t34*t46*t49;
t1168 = Lxcm5*Lycm5*m5*t6*t34*t49;
t1169 = t35*t47*t99;
t1184 = Lx4*m6*t34*t48*t49;
t1185 = Lx4*m6*t40*t46*t49;
t1186 = Lxcm5*Lycm5*m5*t6*t40*t49;
t1187 = t41*t47*t99;
t1188 = Lycm5*Lzcm5*m5*t12*t34*t49;
t1189 = t11*t42*t43*t49;
t1190 = Izz5*t5*t11*t41*t49;
t1191 = Izz6*t5*t11*t41*t49;
t1192 = Lx4*m6*t40*t48*t49;
t1193 = Lycm5*Lzcm5*m5*t12*t40*t49;
t1194 = Lz6*Lzcm6*m6*t3*t4*t35*-2.0;
t1199 = t3*t4*t5*t180;
t1216 = t6*t658;
t1217 = t6*t659;
t1219 = t6*t663;
t1220 = t6*t664;
t1224 = t11*t49*t179*2.0;
t1226 = t3*t10*t11*t179*2.0;
t1227 = t4*t9*t11*t179*2.0;
t1231 = t3*t6*t10*t12*t122;
t1232 = t4*t6*t9*t12*t122;
t1236 = t11*t49*t215*2.0;
t1237 = t11*t49*t221*2.0;
t1238 = t11*t49*t223*2.0;
t1243 = m6*t3*t10*t11*t46*t48*2.0;
t1244 = m6*t4*t9*t11*t46*t48*2.0;
t1245 = m6*t6*t11*t12*t46*t48*2.0;
t1246 = t3*t10*t11*t215*2.0;
t1247 = t4*t9*t11*t215*2.0;
t1248 = t3*t10*t11*t221*2.0;
t1249 = t4*t9*t11*t221*2.0;
t1250 = t3*t10*t11*t223*2.0;
t1251 = t4*t9*t11*t223*2.0;
t1277 = t6*t11*t12*t317;
t1298 = t135+t136;
t1299 = t139+t140;
t1307 = t34*t369*2.0;
t1308 = t34*t370*2.0;
t1309 = t34*t372*2.0;
t1310 = t34*t373*2.0;
t1312 = t36*t372*2.0;
t1313 = t36*t373*2.0;
t1314 = t5*t36*t212*4.0;
t1317 = t35*t395*2.0;
t1318 = t35*t396*2.0;
t1323 = t34*t455*2.0;
t1324 = t34*t456*2.0;
t1345 = -t1007;
t1359 = t3*t4*t867;
t1387 = -t1071;
t1389 = t35*t47*t226;
t1390 = t35*t47*t230;
t1394 = Iyy6*t6*t7*t13*t34*t49;
t1402 = t41*t47*t226;
t1403 = t41*t47*t230;
t1404 = t35*t47*t255;
t1405 = Lz6*m6*t12*t34*t46*t49;
t1406 = t35*t47*t259;
t1407 = Lzcm6*m6*t12*t34*t46*t49;
t1408 = Ixx6*t6*t7*t13*t40*t49;
t1410 = Iyy6*t6*t7*t13*t40*t49;
t1411 = Lz6*m6*t12*t34*t48*t49;
t1412 = Lzcm6*m6*t12*t34*t48*t49;
t1414 = Lz6*m6*t12*t40*t46*t49;
t1416 = Lzcm6*m6*t12*t40*t46*t49;
t1419 = Lz6*m6*t12*t40*t48*t49;
t1420 = Lzcm6*m6*t12*t40*t48*t49;
t1437 = t6*t34*t256*-2.0;
t1438 = t6*t34*t260*-2.0;
t1485 = t35*t658*2.0;
t1486 = t35*t659*2.0;
t1488 = t35*t663*2.0;
t1489 = t35*t664*2.0;
t1492 = t34*t680*2.0;
t1493 = t34*t681*2.0;
t1495 = t35*t711*2.0;
t1497 = t35*t713*2.0;
t1500 = t35*t725*2.0;
t1502 = t35*t727*2.0;
t1506 = t11*t41*t49*t122;
t1534 = t5*t11*t42*t49*t58;
t1558 = t3*t5*t6*t10*t12*t99*2.0;
t1559 = t4*t5*t6*t9*t12*t99*2.0;
t1572 = m6*t34*t35*t46*t48*-2.0;
t1575 = m6*t3*t4*t35*t46*t48*-2.0;
t1590 = Lz6*Lzcm6*m6*t3*t5*t10*t11*t35*-2.0;
t1591 = Lz6*Lzcm6*m6*t4*t5*t9*t11*t35*-2.0;
t1607 = Lxcm6*Lycm6*m6*t6*t34*t36*t49;
t1614 = Lxcm6*Lycm6*m6*t6*t36*t40*t49;
t1615 = Lxcm6*Lycm6*m6*t6*t34*t42*t49;
t1617 = m6*t5*t11*t46*t48*t49*-2.0;
t1621 = m6*t3*t5*t10*t11*t46*t48*-2.0;
t1622 = m6*t4*t5*t9*t11*t46*t48*-2.0;
t1623 = Lxcm6*Lycm6*m6*t6*t40*t42*t49;
t1671 = t34*t36*t372*4.0;
t1672 = t34*t36*t373*4.0;
t1685 = m6*t3*t4*t6*t11*t12*t46*t48*-2.0;
t157 = t5*t111;
t163 = -t104;
t164 = -t112;
t165 = -t113;
t166 = -t114;
t167 = -t115;
t319 = t3*t4*t107;
t322 = t3*t4*t113;
t323 = t3*t4*t115;
t325 = t9*t10*t107;
t330 = -t156;
t341 = t6*t181;
t344 = t6*t185;
t345 = -t158;
t346 = -t159;
t347 = -t160;
t348 = -t162;
t389 = t6*t225;
t397 = t6*t229;
t479 = -t169;
t480 = -t181;
t481 = -t182;
t483 = t5*t146;
t484 = -t185;
t485 = -t186;
t486 = t34*t105;
t487 = t36*t106;
t488 = t35*t107;
t489 = t34*t110;
t490 = t34*t111;
t491 = t36*t110;
t492 = t35*t112;
t493 = t35*t114;
t505 = -t301;
t506 = -t204;
t510 = t5*t150;
t514 = -t225;
t515 = -t227;
t516 = -t229;
t517 = -t231;
t521 = -t241;
t528 = -t316;
t529 = -t254;
t540 = -t265;
t541 = -t267;
t542 = -t268;
t543 = -t270;
t544 = -t271;
t545 = -t272;
t552 = t5*t285;
t553 = t36*t127;
t554 = -t275;
t557 = -t283;
t558 = -t284;
t559 = -t286;
t560 = -t287;
t561 = -t288;
t572 = t3*t4*t126;
t573 = t3*t4*t128;
t587 = t9*t10*t126;
t592 = t9*t10*t128;
t593 = t11*t12*t128;
t608 = -t318;
t609 = -t320;
t610 = -t321;
t619 = -t551;
t621 = t47*t209;
t622 = Lx4*Lz6*m6*t11*t132;
t623 = Lx4*Lzcm5*m5*t11*t132;
t624 = Lx4*Lzcm6*m6*t11*t132;
t633 = t6*t357;
t635 = t6*t360;
t636 = t3*t4*t209;
t639 = t3*t4*t211;
t667 = Ixx5*t11*t12*t132;
t668 = Izz5*t11*t12*t132;
t669 = t11*t45*t134;
t685 = t11*t12*t168;
t689 = Lx4*Lxcm5*m5*t11*t134;
t704 = t6*t438;
t707 = t6*t441;
t718 = t9*t10*t182;
t723 = t9*t10*t184;
t732 = t9*t10*t186;
t744 = t9*t10*t209;
t747 = t9*t10*t211;
t774 = t9*t10*t227;
t781 = t9*t10*t231;
t797 = t3*t4*t145;
t798 = t3*t4*t146;
t803 = -t357;
t804 = -t359;
t805 = -t360;
t806 = t3*t4*t149;
t807 = -t362;
t808 = -t363;
out1 = ft_2({Ixx2,Ixx3,Ixx4,Ixx5,Ixx6,Iyy2,Iyy3,Iyy4,Iyy5,Iyy6,Izz1,Izz2,Izz3,Izz4,Izz5,Izz6,Lx2,Lx3,Lx4,Lxcm1,Lxcm2,Lxcm3,Lxcm4,Lxcm5,Lxcm6,Lycm1,Lycm2,Lycm3,Lycm4,Lycm5,Lycm6,Lz6,Lzcm2,Lzcm3,Lzcm4,Lzcm5,Lzcm6,m1,m2,m3,m4,m5,m6,t10,t1000,t1002,t1003,t1004,t1008,t1009,t1010,t1012,t1013,t1014,t1015,t1016,t1019,t1023,t1026,t103,t1032,t1035,t1038,t104,t1041,t105,t1054,t1055,t1057,t1058,t106,t1061,t107,t1076,t108,t1089,t109,t1090,t1092,t1093,t1099,t11,t110,t1100,t1102,t1103,t1106,t1108,t1109,t111,t1111,t1113,t113,t1136,t1142,t1144,t1146,t115,t1154,t116,t1166,t1167,t1168,t1169,t117,t118,t1184,t1185,t1186,t1187,t1188,t1189,t119,t1190,t1191,t1192,t1193,t1194,t1199,t12,t120,t121,t1216,t1217,t1219,t122,t1220,t1224,t1226,t1227,t1231,t1232,t1236,t1237,t1238,t1243,t1244,t1245,t1246,t1247,t1248,t1249,t125,t1250,t1251,t126,t127,t1277,t128,t129,t1298,t1299,t13,t130,t1307,t1308,t1309,t131,t1310,t1312,t1313,t1314,t1317,t1318,t132,t1323,t1324,t133,t134,t1345,t1359,t137,t1387,t1389,t1390,t1394,t1402,t1403,t1404,t1405,t1406,t1407,t1408,t1410,t1411,t1412,t1414,t1416,t1419,t1420,t1437,t1438,t144,t145,t146,t147,t148,t1485,t1486,t1488,t1489,t149,t1492,t1493,t1495,t1497,t15,t150,t1500,t1502,t1506,t151,t152,t153,t1534,t154,t155,t1558,t1559,t156,t157,t1572,t1575,t1590,t1591,t1607,t161,t1614,t1615,t1617,t162,t1621,t1622,t1623,t163,t164,t165,t166,t167,t1671,t1672,t168,t1685,t17,t170,t171,t172,t173,t174,t175,t176,t177,t178,t179,t180,t181,t185,t187,t188,t189,t19,t190,t192,t193,t198,t199,t2,t205,t206,t209,t211,t212,t213,t214,t215,t217,t218,t219,t220,t221,t223,t225,t226,t228,t229,t230,t232,t233,t234,t237,t238,t240,t242,t243,t244,t246,t248,t250,t252,t253,t255,t257,t259,t265,t266,t269,t270,t271,t272,t273,t274,t276,t277,t278,t279,t280,t281,t282,t283,t284,t285,t288,t289,t290,t291,t292,t293,t294,t295,t296,t297,t298,t299,t3,t300,t302,t303,t304,t305,t306,t307,t308,t309,t310,t311,t312,t313,t314,t319,t320,t321,t322,t323,t324,t325,t326,t327,t33,t330,t331,t332,t333,t334,t335,t336,t337,t338,t339,t34,t340,t341,t344,t345,t346,t347,t348,t349,t35,t351,t352,t354,t355,t358,t359,t36,t361,t362,t363,t365,t366,t367,t368,t371,t372,t373,t374,t375,t376,t377,t379,t380,t381,t382,t383,t384,t385,t386,t387,t388,t389,t390,t392,t393,t394,t397,t398,t399,t4,t40,t400,t401,t404,t405,t406,t407,t408,t409,t41,t410,t411,t412,t42,t420,t421,t422,t423,t425,t426,t428,t429,t43,t431,t432,t435,t436,t438,t439,t44,t440,t441,t443,t444,t445,t446,t447,t448,t449,t45,t450,t451,t454,t457,t458,t459,t46,t460,t461,t462,t463,t464,t466,t467,t468,t47,t470,t471,t473,t475,t476,t477,t478,t479,t48,t480,t481,t482,t483,t484,t485,t486,t487,t488,t489,t49,t490,t491,t492,t493,t494,t495,t496,t497,t498,t499,t5,t50,t500,t501,t502,t503,t504,t505,t506,t507,t508,t509,t51,t510,t511,t512,t513,t514,t515,t516,t517,t518,t519,t52,t520,t521,t522,t523,t524,t525,t526,t527,t528,t529,t53,t530,t531,t532,t533,t534,t535,t536,t537,t538,t539,t54,t540,t541,t542,t543,t544,t545,t546,t547,t548,t549,t55,t550,t552,t553,t554,t555,t556,t557,t558,t559,t56,t560,t561,t562,t563,t564,t565,t566,t567,t568,t569,t57,t570,t571,t572,t573,t575,t576,t577,t578,t579,t58,t580,t585,t586,t587,t588,t589,t59,t590,t591,t592,t593,t594,t595,t596,t597,t598,t599,t6,t60,t600,t601,t602,t603,t608,t609,t61,t610,t612,t613,t614,t615,t619,t62,t620,t621,t622,t623,t624,t629,t63,t630,t631,t632,t633,t634,t635,t636,t637,t638,t639,t64,t640,t641,t642,t643,t645,t646,t647,t648,t65,t650,t651,t652,t653,t655,t656,t657,t66,t661,t662,t666,t667,t668,t669,t67,t670,t671,t672,t674,t675,t676,t677,t678,t679,t68,t682,t685,t686,t687,t688,t689,t69,t690,t692,t693,t694,t695,t697,t699,t7,t70,t700,t701,t702,t704,t706,t707,t708,t709,t71,t710,t711,t712,t713,t714,t715,t716,t717,t718,t719,t72,t721,t723,t724,t725,t726,t727,t728,t729,t73,t730,t731,t732,t733,t734,t735,t736,t737,t738,t74,t740,t741,t742,t743,t744,t747,t748,t749,t75,t750,t752,t753,t754,t755,t756,t757,t759,t76,t760,t761,t762,t763,t764,t766,t767,t768,t769,t77,t770,t771,t772,t773,t774,t775,t776,t777,t778,t779,t78,t780,t781,t782,t783,t784,t785,t787,t789,t79,t790,t791,t792,t793,t794,t795,t797,t798,t8,t80,t800,t801,t802,t803,t804,t805,t806,t807,t808,t809,t81,t815,t816,t825,t826,t831,t832,t834,t835,t836,t837,t838,t839,t840,t841,t842,t843,t844,t845,t847,t848,t85,t852,t857,t86,t861,t862,t863,t864,t867,t87,t870,t871,t872,t873,t874,t875,t88,t883,t884,t885,t886,t887,t89,t894,t895,t896,t9,t90,t908,t909,t910,t911,t912,t913,t917,t918,t919,t92,t920,t921,t923,t927,t928,t929,t93,t930,t931,t932,t933,t934,t935,t936,t937,t938,t94,t941,t942,t943,t944,t96,t97,t971,t975,t976,t977,t981,t982,t983,t984,t985,t986,t99,t999});
end
function out1 = ft_2(ct)
[Ixx2,Ixx3,Ixx4,Ixx5,Ixx6,Iyy2,Iyy3,Iyy4,Iyy5,Iyy6,Izz1,Izz2,Izz3,Izz4,Izz5,Izz6,Lx2,Lx3,Lx4,Lxcm1,Lxcm2,Lxcm3,Lxcm4,Lxcm5,Lxcm6,Lycm1,Lycm2,Lycm3,Lycm4,Lycm5,Lycm6,Lz6,Lzcm2,Lzcm3,Lzcm4,Lzcm5,Lzcm6,m1,m2,m3,m4,m5,m6,t10,t1000,t1002,t1003,t1004,t1008,t1009,t1010,t1012,t1013,t1014,t1015,t1016,t1019,t1023,t1026,t103,t1032,t1035,t1038,t104,t1041,t105,t1054,t1055,t1057,t1058,t106,t1061,t107,t1076,t108,t1089,t109,t1090,t1092,t1093,t1099,t11,t110,t1100,t1102,t1103,t1106,t1108,t1109,t111,t1111,t1113,t113,t1136,t1142,t1144,t1146,t115,t1154,t116,t1166,t1167,t1168,t1169,t117,t118,t1184,t1185,t1186,t1187,t1188,t1189,t119,t1190,t1191,t1192,t1193,t1194,t1199,t12,t120,t121,t1216,t1217,t1219,t122,t1220,t1224,t1226,t1227,t1231,t1232,t1236,t1237,t1238,t1243,t1244,t1245,t1246,t1247,t1248,t1249,t125,t1250,t1251,t126,t127,t1277,t128,t129,t1298,t1299,t13,t130,t1307,t1308,t1309,t131,t1310,t1312,t1313,t1314,t1317,t1318,t132,t1323,t1324,t133,t134,t1345,t1359,t137,t1387,t1389,t1390,t1394,t1402,t1403,t1404,t1405,t1406,t1407,t1408,t1410,t1411,t1412,t1414,t1416,t1419,t1420,t1437,t1438,t144,t145,t146,t147,t148,t1485,t1486,t1488,t1489,t149,t1492,t1493,t1495,t1497,t15,t150,t1500,t1502,t1506,t151,t152,t153,t1534,t154,t155,t1558,t1559,t156,t157,t1572,t1575,t1590,t1591,t1607,t161,t1614,t1615,t1617,t162,t1621,t1622,t1623,t163,t164,t165,t166,t167,t1671,t1672,t168,t1685,t17,t170,t171,t172,t173,t174,t175,t176,t177,t178,t179,t180,t181,t185,t187,t188,t189,t19,t190,t192,t193,t198,t199,t2,t205,t206,t209,t211,t212,t213,t214,t215,t217,t218,t219,t220,t221,t223,t225,t226,t228,t229,t230,t232,t233,t234,t237,t238,t240,t242,t243,t244,t246,t248,t250,t252,t253,t255,t257,t259,t265,t266,t269,t270,t271,t272,t273,t274,t276,t277,t278,t279,t280,t281,t282,t283,t284,t285,t288,t289,t290,t291,t292,t293,t294,t295,t296,t297,t298,t299,t3,t300,t302,t303,t304,t305,t306,t307,t308,t309,t310,t311,t312,t313,t314,t319,t320,t321,t322,t323,t324,t325,t326,t327,t33,t330,t331,t332,t333,t334,t335,t336,t337,t338,t339,t34,t340,t341,t344,t345,t346,t347,t348,t349,t35,t351,t352,t354,t355,t358,t359,t36,t361,t362,t363,t365,t366,t367,t368,t371,t372,t373,t374,t375,t376,t377,t379,t380,t381,t382,t383,t384,t385,t386,t387,t388,t389,t390,t392,t393,t394,t397,t398,t399,t4,t40,t400,t401,t404,t405,t406,t407,t408,t409,t41,t410,t411,t412,t42,t420,t421,t422,t423,t425,t426,t428,t429,t43,t431,t432,t435,t436,t438,t439,t44,t440,t441,t443,t444,t445,t446,t447,t448,t449,t45,t450,t451,t454,t457,t458,t459,t46,t460,t461,t462,t463,t464,t466,t467,t468,t47,t470,t471,t473,t475,t476,t477,t478,t479,t48,t480,t481,t482,t483,t484,t485,t486,t487,t488,t489,t49,t490,t491,t492,t493,t494,t495,t496,t497,t498,t499,t5,t50,t500,t501,t502,t503,t504,t505,t506,t507,t508,t509,t51,t510,t511,t512,t513,t514,t515,t516,t517,t518,t519,t52,t520,t521,t522,t523,t524,t525,t526,t527,t528,t529,t53,t530,t531,t532,t533,t534,t535,t536,t537,t538,t539,t54,t540,t541,t542,t543,t544,t545,t546,t547,t548,t549,t55,t550,t552,t553,t554,t555,t556,t557,t558,t559,t56,t560,t561,t562,t563,t564,t565,t566,t567,t568,t569,t57,t570,t571,t572,t573,t575,t576,t577,t578,t579,t58,t580,t585,t586,t587,t588,t589,t59,t590,t591,t592,t593,t594,t595,t596,t597,t598,t599,t6,t60,t600,t601,t602,t603,t608,t609,t61,t610,t612,t613,t614,t615,t619,t62,t620,t621,t622,t623,t624,t629,t63,t630,t631,t632,t633,t634,t635,t636,t637,t638,t639,t64,t640,t641,t642,t643,t645,t646,t647,t648,t65,t650,t651,t652,t653,t655,t656,t657,t66,t661,t662,t666,t667,t668,t669,t67,t670,t671,t672,t674,t675,t676,t677,t678,t679,t68,t682,t685,t686,t687,t688,t689,t69,t690,t692,t693,t694,t695,t697,t699,t7,t70,t700,t701,t702,t704,t706,t707,t708,t709,t71,t710,t711,t712,t713,t714,t715,t716,t717,t718,t719,t72,t721,t723,t724,t725,t726,t727,t728,t729,t73,t730,t731,t732,t733,t734,t735,t736,t737,t738,t74,t740,t741,t742,t743,t744,t747,t748,t749,t75,t750,t752,t753,t754,t755,t756,t757,t759,t76,t760,t761,t762,t763,t764,t766,t767,t768,t769,t77,t770,t771,t772,t773,t774,t775,t776,t777,t778,t779,t78,t780,t781,t782,t783,t784,t785,t787,t789,t79,t790,t791,t792,t793,t794,t795,t797,t798,t8,t80,t800,t801,t802,t803,t804,t805,t806,t807,t808,t809,t81,t815,t816,t825,t826,t831,t832,t834,t835,t836,t837,t838,t839,t840,t841,t842,t843,t844,t845,t847,t848,t85,t852,t857,t86,t861,t862,t863,t864,t867,t87,t870,t871,t872,t873,t874,t875,t88,t883,t884,t885,t886,t887,t89,t894,t895,t896,t9,t90,t908,t909,t910,t911,t912,t913,t917,t918,t919,t92,t920,t921,t923,t927,t928,t929,t93,t930,t931,t932,t933,t934,t935,t936,t937,t938,t94,t941,t942,t943,t944,t96,t97,t971,t975,t976,t977,t981,t982,t983,t984,t985,t986,t99,t999] = ct{:};
t810 = -t365;
t811 = -t562;
t812 = t5*t6*t149;
t813 = -t563;
t814 = -t367;
t817 = t3*t4*t150;
t818 = -t564;
t819 = -t566;
t820 = t3*t4*t151;
t822 = -t390;
t823 = -t570;
t824 = t3*t4*t152;
t828 = -t398;
t829 = -t571;
t830 = -t399;
t833 = -t406;
t846 = -t436;
t849 = -t438;
t850 = -t440;
t851 = -t441;
t853 = -t443;
t854 = -t444;
t855 = -t445;
t856 = -t446;
t858 = -t575;
t859 = -t448;
t860 = -t451;
t865 = -t577;
t866 = -t459;
t868 = t11*t12*t149;
t869 = -t466;
t876 = -t475;
t877 = -t477;
t878 = -t478;
t888 = t3*t10*t11*t107;
t889 = t4*t9*t11*t107;
t890 = t6*t11*t12*t107;
t891 = t3*t10*t11*t111;
t892 = t4*t9*t11*t111;
t893 = t6*t11*t12*t111;
t897 = t9*t10*t278;
t899 = t36*t265;
t900 = t9*t10*t288;
t901 = t9*t10*t289;
t902 = t35*t270;
t903 = t35*t271;
t904 = t35*t272;
t905 = t6*t338*2.0;
t907 = t6*t361*2.0;
t914 = t6*t445*2.0;
t915 = t11*t12*t181*2.0;
t916 = t11*t12*t185*2.0;
t922 = t6*t463*2.0;
t924 = t11*t12*t225*2.0;
t926 = t11*t12*t229*2.0;
t939 = t5*t589;
t940 = t7*t11*t13*t126;
t945 = t3*t10*t12*t127;
t946 = t4*t9*t12*t127;
t947 = t7*t12*t13*t127;
t948 = t7*t11*t13*t128;
t949 = t3*t10*t11*t129;
t950 = t4*t9*t11*t129;
t951 = t3*t10*t11*t130;
t952 = t4*t9*t11*t130;
t953 = t3*t10*t11*t131;
t954 = t4*t9*t11*t131;
t956 = t34*t283;
t957 = t36*t284;
t958 = t35*t285;
t959 = t34*t288;
t960 = t34*t289;
t961 = t36*t288;
t962 = t35*t290;
t963 = t35*t292;
t964 = t35*t294;
t967 = -t594;
t968 = -t597;
t969 = -t602;
t970 = -t603;
t973 = t884*2.0;
t974 = t885*2.0;
t978 = t886*2.0;
t979 = t887*2.0;
t980 = t36*t211*2.0;
t987 = t3*t4*t283;
t988 = t3*t4*t285;
t989 = t3*t4*t288;
t990 = t3*t4*t289;
t991 = t3*t4*t291;
t992 = t3*t4*t293;
t993 = t3*t4*t295;
t994 = t40*t497;
t995 = t40*t498;
t996 = t40*t507;
t997 = t40*t508;
t1001 = t5*t679;
t1005 = t11*t81*t134;
t1006 = t6*t700;
t1011 = t11*t12*t338;
t1017 = t3*t10*t12*t181;
t1020 = t4*t9*t12*t181;
t1024 = t3*t10*t12*t185;
t1027 = t4*t9*t12*t185;
t1036 = t6*t737;
t1044 = t3*t10*t12*t225;
t1046 = t4*t9*t12*t225;
t1049 = t3*t10*t12*t229;
t1051 = t4*t9*t12*t229;
t1056 = t9*t10*t406;
t1060 = t6*t791;
t1070 = t36*t320;
t1072 = t11*t12*t463;
t1077 = -t629;
t1078 = -t632;
t1080 = -t634;
t1084 = -t640;
t1085 = -t641;
t1086 = t3*t4*t511;
t1087 = t3*t4*t512;
t1088 = t3*t4*t513;
t1096 = -t670;
t1097 = t3*t4*t519;
t1098 = -t676;
t1101 = -t911;
t1104 = -t686;
t1105 = -t687;
t1107 = -t694;
t1110 = -t700;
t1115 = -t708;
t1116 = -t709;
t1118 = t3*t4*t530;
t1119 = -t712;
t1120 = -t714;
t1121 = t3*t4*t531;
t1122 = -t716;
t1123 = -t717;
t1125 = t3*t10*t11*t146;
t1126 = t4*t9*t11*t146;
t1127 = t3*t4*t533;
t1128 = -t726;
t1129 = -t728;
t1130 = t3*t4*t534;
t1131 = -t730;
t1132 = -t731;
t1138 = t3*t10*t11*t150;
t1139 = t4*t9*t11*t150;
t1140 = -t923;
t1141 = -t750;
t1143 = -t757;
t1145 = -t764;
t1147 = -t769;
t1148 = -t770;
t1149 = -t771;
t1150 = -t772;
t1151 = -t773;
t1152 = -t775;
t1155 = -t776;
t1156 = -t777;
t1157 = -t778;
t1158 = -t779;
t1159 = -t780;
t1160 = -t782;
t1162 = t7*t12*t13*t154;
t1163 = -t787;
t1165 = -t790;
t1170 = t5*t11*t49*t105;
t1172 = t3*t5*t10*t11*t105;
t1173 = t4*t5*t9*t11*t105;
t1176 = t3*t5*t10*t11*t110;
t1177 = t4*t5*t9*t11*t110;
t1180 = t3*t5*t10*t11*t113;
t1181 = t4*t5*t9*t11*t113;
t1182 = t3*t5*t10*t11*t115;
t1183 = t4*t5*t9*t11*t115;
t1202 = -t977;
t1203 = -t981;
t1204 = -t982;
t1205 = -t984;
t1206 = -t986;
t1207 = m6*t33*t273;
t1221 = -t894;
t1222 = t7*t13*t43*t134;
t1223 = Iyy6*t5*t7*t13*t134;
t1239 = t11*t12*t57*t132;
t1240 = t11*t12*t62*t132;
t1241 = t11*t12*t65*t132;
t1242 = t11*t12*t66*t132;
t1254 = t3*t4*t588;
t1255 = t3*t6*t10*t12*t125;
t1256 = t4*t6*t9*t12*t125;
t1257 = t7*t12*t13*t309;
t1258 = t3*t7*t10*t13*t126;
t1259 = t4*t7*t9*t13*t126;
t1264 = t3*t7*t10*t13*t128;
t1265 = t4*t7*t9*t13*t128;
t1266 = t6*t11*t12*t312;
t1267 = t3*t6*t10*t12*t129;
t1268 = t4*t6*t9*t12*t129;
t1269 = t6*t11*t12*t313;
t1270 = t3*t6*t10*t12*t130;
t1271 = t4*t6*t9*t12*t130;
t1272 = t6*t11*t12*t314;
t1273 = t3*t6*t10*t12*t131;
t1274 = t4*t6*t9*t12*t131;
t1275 = t9*t10*t576;
t1276 = t9*t10*t578;
t1278 = t9*t10*t588;
t1281 = t9*t10*t594;
t1282 = t6*t11*t12*t270;
t1283 = t6*t11*t12*t271;
t1284 = t6*t11*t12*t272;
t1285 = -t921;
t1286 = -t935;
t1287 = -t936;
t1288 = -t937;
t1289 = -t938;
t1291 = -t941;
t1292 = -t942;
t1293 = -t943;
t1294 = -t944;
t1305 = t34*t362*2.0;
t1306 = t34*t363*2.0;
t1311 = t36*t371*2.0;
t1315 = t34*t570;
t1316 = t35*t394*2.0;
t1319 = t34*t571;
t1320 = t34*t443*2.0;
t1321 = t34*t444*2.0;
t1326 = t36*t467*2.0;
t1327 = t35*t477*2.0;
t1328 = t3*t10*t11*t285;
t1329 = t4*t9*t11*t285;
t1330 = t11*t12*t36*t126;
t1331 = t3*t10*t11*t289;
t1332 = t4*t9*t11*t289;
t1338 = t3*t4*t570;
t1339 = t3*t4*t571;
t1341 = -t999;
t1342 = -t1000;
t1343 = Lz6*Lzcm6*m6*t11*t12*t132*-2.0;
t1346 = -t1010;
t1347 = -t1012;
t1348 = -t1014;
t1349 = -t1016;
t1351 = -t1019;
t1353 = t6*t715*-2.0;
t1354 = -t1023;
t1356 = -t1026;
t1358 = t6*t729*-2.0;
t1360 = t11*t49*t504;
t1361 = t11*t134*t149;
t1362 = t3*t10*t11*t504;
t1363 = t4*t9*t11*t504;
t1365 = t3*t6*t10*t11*t149;
t1367 = t4*t6*t9*t11*t149;
t1369 = -t1243;
t1370 = -t1244;
t1371 = -t1245;
t1374 = t6*t775*-2.0;
t1377 = t6*t782*-2.0;
t1379 = t6*t7*t11*t13*t127*2.0;
t1380 = -t1054;
t1381 = -t1055;
t1388 = t36*t47*t211;
t1391 = t35*t36*t154;
t1392 = t11*t12*t107*t132;
t1393 = t6*t7*t13*t49*t106;
t1396 = t3*t6*t10*t12*t156;
t1397 = t4*t6*t9*t12*t156;
t1398 = t6*t11*t12*t321;
t1409 = Iyy6*t11*t12*t42*t132;
t1421 = -t1169;
t1422 = -t1309;
t1423 = -t1310;
t1424 = -t1312;
t1425 = -t1313;
t1426 = -t1314;
t1435 = -t1185;
t1436 = -t1186;
t1439 = -t1190;
t1440 = -t1191;
t1441 = -t1192;
t1442 = -t1193;
t1452 = t3*t4*t5*t504;
t1474 = t134+t274;
t1481 = t36*t640*2.0;
t1482 = t36*t641*2.0;
t1484 = t35*t657*2.0;
t1487 = t35*t662*2.0;
t1490 = t3*t6*t7*t10*t13*t106*2.0;
t1491 = t4*t6*t7*t9*t13*t106*2.0;
t1494 = t35*t710*2.0;
t1496 = t34*t716*2.0;
t1498 = t34*t717*2.0;
t1499 = t35*t724*2.0;
t1501 = t34*t730*2.0;
t1503 = t34*t731*2.0;
t1507 = t133+t296;
t1508 = t11*t35*t49*t125;
t1510 = t3*t10*t11*t547;
t1511 = t4*t9*t11*t547;
t1513 = t35*t923;
t1514 = t34*t772*2.0;
t1515 = t34*t773*2.0;
t1516 = t35*t771*2.0;
t1517 = t34*t779*2.0;
t1518 = t34*t780*2.0;
t1519 = t35*t778*2.0;
t1520 = t3*t10*t11*t35*t125;
t1521 = t4*t9*t11*t35*t125;
t1524 = t3*t10*t11*t35*t127;
t1525 = t4*t9*t11*t35*t127;
t1535 = t11*t41*t49*t129;
t1536 = t11*t41*t49*t130;
t1537 = t11*t41*t49*t131;
t1538 = t35*t792*2.0;
t1539 = t35*t794*2.0;
t1540 = t137+t297;
t1543 = t11*t81*t274*2.0;
t1544 = t3*t10*t11*t340*2.0;
t1545 = t4*t9*t11*t340*2.0;
t1549 = t11*t88*t274*2.0;
t1551 = t12*t99*t274*2.0;
t1552 = t5*t7*t13*t58*t134;
t1553 = t7*t13*t127*t134;
t1554 = t3*t10*t11*t366*2.0;
t1555 = t4*t9*t11*t366*2.0;
t1564 = t3*t6*t7*t10*t13*t127;
t1565 = t4*t6*t7*t9*t13*t127;
t1566 = t3*t7*t10*t13*t266;
t1567 = t4*t7*t9*t13*t266;
t1569 = t3*t7*t10*t13*t269;
t1570 = t4*t7*t9*t13*t269;
t1573 = -t1389;
t1574 = -t1390;
t1586 = -t1495;
t1587 = -t1497;
t1588 = -t1500;
t1589 = -t1502;
t1593 = -t1410;
t1594 = t41*t47*t530;
t1595 = -t1414;
t1596 = t41*t47*t533;
t1597 = -t1416;
t1599 = t6*t11*t12*t36*t154;
t1600 = -t1419;
t1601 = -t1420;
t1604 = t6*t1298;
t1605 = t12*t1298;
t1606 = t6*t1299;
t1608 = t12*t1299;
t1618 = t5*t11*t42*t49*t110;
t1628 = t11*t36*t126*t134;
t1629 = t7*t13*t34*t49*t126;
t1630 = t7*t13*t34*t49*t128;
t1632 = t3*t5*t10*t12*t36*t126;
t1633 = t4*t5*t9*t12*t36*t126;
t1637 = t7*t13*t40*t49*t126;
t1638 = t11*t42*t128*t134;
t1639 = t7*t13*t40*t49*t128;
t1652 = m6*t11*t12*t46*t48*t132*2.0;
t1653 = t12*t226*t274*2.0;
t1654 = t12*t230*t274*2.0;
t1656 = t3*t6*t10*t12*t566;
t1657 = t4*t6*t9*t12*t566;
t1658 = t3*t5*t10*t12*t390*2.0;
t1659 = t4*t5*t9*t12*t390*2.0;
t1660 = t3*t5*t10*t12*t398*2.0;
t1661 = t4*t5*t9*t12*t398*2.0;
t1662 = -t1534;
t1663 = t12*t255*t274*2.0;
t1664 = t12*t259*t274*2.0;
t1665 = t3*t5*t10*t12*t450*2.0;
t1666 = t4*t5*t9*t12*t450*2.0;
t1667 = t3*t5*t10*t12*t458*2.0;
t1668 = t4*t5*t9*t12*t458*2.0;
t1669 = t6*t11*t12*t923;
t1699 = -t1614;
t1700 = -t1615;
t1716 = t11*t35*t42*t49*t127;
t1720 = t35*t1617;
t1721 = t35*t1621;
t1722 = t35*t1622;
t1741 = t45+t81+t126+t128+t149+t228+t232+t531+t534;
t625 = -t325;
t626 = t9*t10*t165;
t627 = t9*t10*t167;
t796 = -t341;
t799 = -t344;
t821 = -t389;
t827 = -t397;
t879 = -t486;
t880 = -t487;
t881 = -t489;
t882 = -t491;
t906 = -t553;
t965 = -t587;
t966 = -t592;
t1022 = t9*t10*t341;
t1029 = t9*t10*t344;
t1048 = t9*t10*t389;
t1053 = t9*t10*t397;
t1065 = t47*t483;
t1066 = t3*t4*t481;
t1067 = t3*t4*t483;
t1068 = t3*t4*t485;
t1069 = t35*t319;
t1073 = -t622;
t1074 = -t623;
t1075 = -t624;
t1079 = -t633;
t1081 = -t635;
t1082 = -t907;
t1083 = t3*t4*t510;
t1091 = t3*t4*t515;
t1094 = t3*t4*t517;
t1095 = -t667;
t1112 = -t704;
t1114 = -t707;
t1117 = -t914;
t1124 = -t915;
t1133 = -t916;
t1134 = t35*t325;
t1137 = -t744;
t1153 = -t924;
t1161 = -t926;
t1164 = t11*t12*t521;
t1171 = t11*t49*t157;
t1178 = t3*t10*t11*t157;
t1179 = t4*t9*t11*t157;
t1196 = t36*t489;
t1210 = -t888;
t1211 = -t889;
t1212 = -t890;
t1233 = t9*t10*t557;
t1234 = t9*t10*t561;
t1235 = -t901;
t1260 = t11*t12*t573;
t1261 = t6*t945;
t1262 = t6*t946;
t1280 = t11*t12*t592;
t1290 = -t940;
t1295 = -t945;
t1296 = -t946;
t1297 = -t947;
t1300 = -t958;
t1301 = -t960;
t1302 = -t962;
t1303 = -t963;
t1304 = -t964;
t1333 = t36*t593;
t1334 = -t988;
t1335 = -t991;
t1336 = -t992;
t1337 = -t993;
t1340 = t3*t4*t833;
t1344 = -t1006;
t1350 = t3*t10*t11*t481;
t1352 = t4*t9*t11*t481;
t1355 = t3*t10*t11*t485;
t1357 = t4*t9*t11*t485;
t1364 = t11*t12*t806;
t1366 = t11*t12*t807;
t1368 = t11*t12*t808;
t1372 = t3*t10*t11*t515;
t1373 = t4*t9*t11*t515;
t1375 = t3*t10*t11*t517;
t1376 = t4*t9*t11*t517;
t1378 = t5*t940*2.0;
t1382 = t5*t1162;
t1383 = t11*t12*t853;
t1384 = t11*t12*t854;
t1385 = t11*t12*t855;
t1395 = t6*t11*t12*t319;
t1399 = t3*t6*t10*t12*t157;
t1400 = t4*t6*t9*t12*t157;
t1417 = t6*t11*t12*t325;
t1427 = -t1316;
t1428 = -t1170;
t1429 = -t1172;
t1430 = -t1173;
t1431 = t3*t10*t11*t330;
t1432 = t4*t9*t11*t330;
t1433 = -t1176;
t1434 = -t1177;
t1443 = -t1326;
t1445 = t132*t480;
t1446 = t132*t484;
t1449 = -t1207;
t1450 = t132*t514;
t1451 = t132*t516;
t1453 = t6*t1077;
t1456 = -t1222;
t1458 = t3*t4*t958;
t1460 = -t1240;
t1461 = -t1241;
t1462 = -t1242;
t1463 = -t1255;
t1464 = -t1256;
out1 = ft_3({Ixx2,Ixx3,Ixx4,Ixx5,Ixx6,Iyy2,Iyy3,Iyy4,Iyy5,Iyy6,Izz1,Izz2,Izz3,Izz4,Izz5,Izz6,Lx2,Lx3,Lx4,Lxcm1,Lxcm2,Lxcm3,Lxcm4,Lxcm5,Lxcm6,Lycm1,Lycm2,Lycm3,Lycm4,Lycm5,Lycm6,Lz6,Lzcm2,Lzcm3,Lzcm4,Lzcm5,Lzcm6,m1,m2,m3,m4,m5,m6,t10,t1001,t1002,t1003,t1004,t1005,t1008,t1009,t1011,t1013,t1015,t1017,t1020,t1022,t1024,t1027,t1029,t103,t1032,t1035,t1036,t1038,t104,t1041,t1044,t1046,t1048,t1049,t105,t1051,t1053,t1056,t1057,t1058,t106,t1060,t1061,t1065,t1066,t1067,t1068,t1069,t107,t1070,t1072,t1073,t1074,t1075,t1076,t1077,t1078,t1079,t108,t1080,t1081,t1082,t1083,t1084,t1085,t1086,t1087,t1088,t1089,t109,t1090,t1091,t1092,t1093,t1094,t1095,t1096,t1097,t1098,t1099,t11,t110,t1100,t1101,t1102,t1103,t1104,t1105,t1106,t1107,t1108,t1109,t111,t1110,t1111,t1112,t1113,t1114,t1115,t1116,t1117,t1118,t1119,t1120,t1121,t1122,t1123,t1124,t1125,t1126,t1127,t1128,t1129,t113,t1130,t1131,t1132,t1133,t1134,t1136,t1137,t1138,t1139,t1140,t1141,t1142,t1143,t1144,t1145,t1146,t1147,t1148,t1149,t115,t1150,t1151,t1152,t1153,t1154,t1155,t1156,t1157,t1158,t1159,t116,t1160,t1161,t1162,t1163,t1164,t1165,t1166,t1167,t1168,t117,t1171,t1178,t1179,t118,t1180,t1181,t1182,t1183,t1184,t1187,t1188,t1189,t119,t1194,t1196,t1199,t12,t120,t1202,t1203,t1204,t1205,t1206,t121,t1210,t1211,t1212,t1216,t1217,t1219,t122,t1220,t1221,t1223,t1224,t1226,t1227,t1231,t1232,t1233,t1234,t1235,t1236,t1237,t1238,t1239,t1246,t1247,t1248,t1249,t125,t1250,t1251,t1254,t1257,t1258,t1259,t1260,t1261,t1262,t1264,t1265,t1266,t1267,t1268,t1269,t127,t1270,t1271,t1272,t1273,t1274,t1275,t1276,t1277,t1278,t1280,t1281,t1282,t1283,t1284,t1285,t1286,t1287,t1288,t1289,t129,t1290,t1291,t1292,t1293,t1294,t1295,t1296,t1297,t1298,t1299,t13,t130,t1300,t1301,t1302,t1303,t1304,t1305,t1306,t1307,t1308,t131,t1311,t1315,t1317,t1318,t1319,t132,t1320,t1321,t1323,t1324,t1327,t1328,t1329,t1330,t1331,t1332,t1333,t1334,t1335,t1336,t1337,t1338,t1339,t1340,t1341,t1342,t1343,t1344,t1345,t1346,t1347,t1348,t1349,t1350,t1351,t1352,t1353,t1354,t1355,t1356,t1357,t1358,t1359,t1360,t1361,t1362,t1363,t1364,t1365,t1366,t1367,t1368,t1369,t1370,t1371,t1372,t1373,t1374,t1375,t1376,t1377,t1378,t1379,t1380,t1381,t1382,t1383,t1384,t1385,t1387,t1388,t1391,t1392,t1393,t1394,t1395,t1396,t1397,t1398,t1399,t1400,t1402,t1403,t1404,t1405,t1406,t1407,t1408,t1409,t1411,t1412,t1417,t1421,t1422,t1423,t1424,t1425,t1426,t1427,t1428,t1429,t1430,t1431,t1432,t1433,t1434,t1435,t1436,t1437,t1438,t1439,t144,t1440,t1441,t1442,t1443,t1445,t1446,t1449,t145,t1450,t1451,t1452,t1453,t1456,t1458,t146,t1460,t1461,t1462,t1463,t1464,t147,t1474,t148,t1481,t1482,t1484,t1485,t1486,t1487,t1488,t1489,t1490,t1491,t1492,t1493,t1494,t1496,t1498,t1499,t15,t150,t1501,t1503,t1506,t1507,t1508,t151,t1510,t1511,t1513,t1514,t1515,t1516,t1517,t1518,t1519,t152,t1520,t1521,t1524,t1525,t153,t1535,t1536,t1537,t1538,t1539,t154,t1540,t1543,t1544,t1545,t1549,t155,t1551,t1552,t1553,t1554,t1555,t1558,t1559,t1564,t1565,t1566,t1567,t1569,t157,t1570,t1572,t1573,t1574,t1575,t1586,t1587,t1588,t1589,t1590,t1591,t1593,t1594,t1595,t1596,t1597,t1599,t1600,t1601,t1604,t1605,t1606,t1607,t1608,t161,t1617,t1618,t162,t1621,t1622,t1623,t1628,t1629,t163,t1630,t1632,t1633,t1637,t1638,t1639,t164,t165,t1652,t1653,t1654,t1656,t1657,t1658,t1659,t166,t1660,t1661,t1662,t1663,t1664,t1665,t1666,t1667,t1668,t1669,t167,t1671,t1672,t168,t1685,t1699,t17,t170,t1700,t171,t1716,t172,t1720,t1721,t1722,t173,t174,t1741,t175,t176,t177,t178,t179,t180,t187,t188,t189,t19,t190,t192,t193,t198,t199,t2,t205,t206,t209,t212,t213,t214,t215,t217,t218,t219,t220,t221,t223,t226,t230,t233,t234,t237,t238,t240,t242,t243,t244,t246,t248,t250,t252,t253,t257,t266,t269,t276,t277,t278,t279,t280,t281,t282,t283,t285,t288,t289,t290,t291,t292,t293,t294,t295,t298,t299,t3,t300,t302,t303,t304,t305,t306,t307,t308,t309,t310,t311,t312,t313,t314,t319,t322,t323,t324,t326,t327,t330,t331,t332,t333,t334,t335,t336,t337,t338,t339,t34,t340,t345,t346,t347,t348,t349,t35,t351,t352,t354,t355,t358,t359,t36,t368,t372,t373,t374,t375,t376,t377,t379,t380,t381,t382,t383,t384,t385,t386,t387,t388,t392,t393,t394,t4,t40,t400,t401,t404,t405,t407,t408,t409,t410,t411,t412,t42,t420,t421,t422,t423,t425,t426,t428,t429,t43,t431,t432,t435,t439,t44,t440,t447,t449,t450,t454,t457,t458,t460,t461,t462,t463,t464,t467,t468,t47,t470,t471,t473,t476,t479,t480,t481,t482,t483,t484,t485,t488,t49,t490,t491,t492,t493,t494,t495,t496,t497,t498,t499,t5,t50,t500,t501,t502,t503,t504,t505,t506,t507,t508,t509,t51,t510,t511,t512,t513,t514,t515,t516,t517,t518,t519,t52,t520,t521,t522,t523,t524,t525,t526,t527,t528,t529,t53,t530,t532,t533,t535,t536,t537,t538,t539,t54,t540,t541,t542,t543,t544,t545,t546,t547,t548,t549,t55,t550,t552,t553,t554,t555,t556,t557,t558,t559,t56,t560,t561,t565,t567,t568,t569,t57,t570,t571,t572,t573,t576,t578,t579,t58,t580,t585,t586,t588,t589,t59,t590,t591,t593,t595,t596,t598,t599,t6,t60,t600,t601,t608,t609,t61,t610,t612,t613,t614,t615,t619,t62,t620,t621,t625,t626,t627,t63,t630,t631,t634,t636,t637,t638,t639,t64,t642,t643,t645,t646,t647,t648,t65,t650,t651,t652,t653,t655,t656,t657,t66,t661,t662,t666,t668,t669,t67,t671,t672,t674,t675,t677,t678,t679,t68,t682,t685,t688,t689,t69,t690,t692,t693,t695,t697,t699,t7,t70,t701,t702,t706,t71,t711,t713,t718,t719,t72,t721,t723,t725,t727,t73,t732,t733,t734,t735,t736,t737,t738,t74,t740,t741,t742,t743,t747,t748,t749,t75,t752,t753,t754,t755,t756,t759,t76,t760,t761,t762,t763,t766,t767,t768,t77,t774,t78,t781,t783,t784,t785,t789,t79,t791,t792,t793,t794,t795,t796,t797,t798,t799,t8,t80,t800,t801,t802,t803,t804,t805,t806,t807,t808,t809,t81,t810,t811,t812,t813,t814,t815,t816,t817,t818,t819,t820,t821,t822,t823,t824,t825,t826,t827,t828,t829,t830,t831,t832,t833,t834,t835,t836,t837,t838,t839,t840,t841,t842,t843,t844,t845,t846,t847,t848,t849,t85,t850,t851,t852,t853,t854,t855,t856,t857,t858,t859,t86,t860,t861,t862,t863,t864,t865,t866,t867,t868,t869,t87,t870,t871,t872,t873,t874,t875,t876,t877,t878,t879,t88,t880,t881,t882,t883,t884,t885,t886,t887,t89,t891,t892,t893,t895,t896,t897,t899,t9,t90,t900,t902,t903,t904,t905,t906,t908,t909,t910,t912,t913,t917,t918,t919,t92,t920,t922,t927,t928,t929,t93,t930,t931,t932,t933,t934,t939,t94,t947,t948,t949,t950,t951,t952,t953,t954,t956,t957,t958,t959,t96,t961,t965,t966,t967,t968,t969,t97,t970,t971,t973,t974,t975,t976,t978,t979,t980,t983,t985,t987,t989,t99,t990,t994,t995,t996,t997});
end
function out1 = ft_3(ct)
[Ixx2,Ixx3,Ixx4,Ixx5,Ixx6,Iyy2,Iyy3,Iyy4,Iyy5,Iyy6,Izz1,Izz2,Izz3,Izz4,Izz5,Izz6,Lx2,Lx3,Lx4,Lxcm1,Lxcm2,Lxcm3,Lxcm4,Lxcm5,Lxcm6,Lycm1,Lycm2,Lycm3,Lycm4,Lycm5,Lycm6,Lz6,Lzcm2,Lzcm3,Lzcm4,Lzcm5,Lzcm6,m1,m2,m3,m4,m5,m6,t10,t1001,t1002,t1003,t1004,t1005,t1008,t1009,t1011,t1013,t1015,t1017,t1020,t1022,t1024,t1027,t1029,t103,t1032,t1035,t1036,t1038,t104,t1041,t1044,t1046,t1048,t1049,t105,t1051,t1053,t1056,t1057,t1058,t106,t1060,t1061,t1065,t1066,t1067,t1068,t1069,t107,t1070,t1072,t1073,t1074,t1075,t1076,t1077,t1078,t1079,t108,t1080,t1081,t1082,t1083,t1084,t1085,t1086,t1087,t1088,t1089,t109,t1090,t1091,t1092,t1093,t1094,t1095,t1096,t1097,t1098,t1099,t11,t110,t1100,t1101,t1102,t1103,t1104,t1105,t1106,t1107,t1108,t1109,t111,t1110,t1111,t1112,t1113,t1114,t1115,t1116,t1117,t1118,t1119,t1120,t1121,t1122,t1123,t1124,t1125,t1126,t1127,t1128,t1129,t113,t1130,t1131,t1132,t1133,t1134,t1136,t1137,t1138,t1139,t1140,t1141,t1142,t1143,t1144,t1145,t1146,t1147,t1148,t1149,t115,t1150,t1151,t1152,t1153,t1154,t1155,t1156,t1157,t1158,t1159,t116,t1160,t1161,t1162,t1163,t1164,t1165,t1166,t1167,t1168,t117,t1171,t1178,t1179,t118,t1180,t1181,t1182,t1183,t1184,t1187,t1188,t1189,t119,t1194,t1196,t1199,t12,t120,t1202,t1203,t1204,t1205,t1206,t121,t1210,t1211,t1212,t1216,t1217,t1219,t122,t1220,t1221,t1223,t1224,t1226,t1227,t1231,t1232,t1233,t1234,t1235,t1236,t1237,t1238,t1239,t1246,t1247,t1248,t1249,t125,t1250,t1251,t1254,t1257,t1258,t1259,t1260,t1261,t1262,t1264,t1265,t1266,t1267,t1268,t1269,t127,t1270,t1271,t1272,t1273,t1274,t1275,t1276,t1277,t1278,t1280,t1281,t1282,t1283,t1284,t1285,t1286,t1287,t1288,t1289,t129,t1290,t1291,t1292,t1293,t1294,t1295,t1296,t1297,t1298,t1299,t13,t130,t1300,t1301,t1302,t1303,t1304,t1305,t1306,t1307,t1308,t131,t1311,t1315,t1317,t1318,t1319,t132,t1320,t1321,t1323,t1324,t1327,t1328,t1329,t1330,t1331,t1332,t1333,t1334,t1335,t1336,t1337,t1338,t1339,t1340,t1341,t1342,t1343,t1344,t1345,t1346,t1347,t1348,t1349,t1350,t1351,t1352,t1353,t1354,t1355,t1356,t1357,t1358,t1359,t1360,t1361,t1362,t1363,t1364,t1365,t1366,t1367,t1368,t1369,t1370,t1371,t1372,t1373,t1374,t1375,t1376,t1377,t1378,t1379,t1380,t1381,t1382,t1383,t1384,t1385,t1387,t1388,t1391,t1392,t1393,t1394,t1395,t1396,t1397,t1398,t1399,t1400,t1402,t1403,t1404,t1405,t1406,t1407,t1408,t1409,t1411,t1412,t1417,t1421,t1422,t1423,t1424,t1425,t1426,t1427,t1428,t1429,t1430,t1431,t1432,t1433,t1434,t1435,t1436,t1437,t1438,t1439,t144,t1440,t1441,t1442,t1443,t1445,t1446,t1449,t145,t1450,t1451,t1452,t1453,t1456,t1458,t146,t1460,t1461,t1462,t1463,t1464,t147,t1474,t148,t1481,t1482,t1484,t1485,t1486,t1487,t1488,t1489,t1490,t1491,t1492,t1493,t1494,t1496,t1498,t1499,t15,t150,t1501,t1503,t1506,t1507,t1508,t151,t1510,t1511,t1513,t1514,t1515,t1516,t1517,t1518,t1519,t152,t1520,t1521,t1524,t1525,t153,t1535,t1536,t1537,t1538,t1539,t154,t1540,t1543,t1544,t1545,t1549,t155,t1551,t1552,t1553,t1554,t1555,t1558,t1559,t1564,t1565,t1566,t1567,t1569,t157,t1570,t1572,t1573,t1574,t1575,t1586,t1587,t1588,t1589,t1590,t1591,t1593,t1594,t1595,t1596,t1597,t1599,t1600,t1601,t1604,t1605,t1606,t1607,t1608,t161,t1617,t1618,t162,t1621,t1622,t1623,t1628,t1629,t163,t1630,t1632,t1633,t1637,t1638,t1639,t164,t165,t1652,t1653,t1654,t1656,t1657,t1658,t1659,t166,t1660,t1661,t1662,t1663,t1664,t1665,t1666,t1667,t1668,t1669,t167,t1671,t1672,t168,t1685,t1699,t17,t170,t1700,t171,t1716,t172,t1720,t1721,t1722,t173,t174,t1741,t175,t176,t177,t178,t179,t180,t187,t188,t189,t19,t190,t192,t193,t198,t199,t2,t205,t206,t209,t212,t213,t214,t215,t217,t218,t219,t220,t221,t223,t226,t230,t233,t234,t237,t238,t240,t242,t243,t244,t246,t248,t250,t252,t253,t257,t266,t269,t276,t277,t278,t279,t280,t281,t282,t283,t285,t288,t289,t290,t291,t292,t293,t294,t295,t298,t299,t3,t300,t302,t303,t304,t305,t306,t307,t308,t309,t310,t311,t312,t313,t314,t319,t322,t323,t324,t326,t327,t330,t331,t332,t333,t334,t335,t336,t337,t338,t339,t34,t340,t345,t346,t347,t348,t349,t35,t351,t352,t354,t355,t358,t359,t36,t368,t372,t373,t374,t375,t376,t377,t379,t380,t381,t382,t383,t384,t385,t386,t387,t388,t392,t393,t394,t4,t40,t400,t401,t404,t405,t407,t408,t409,t410,t411,t412,t42,t420,t421,t422,t423,t425,t426,t428,t429,t43,t431,t432,t435,t439,t44,t440,t447,t449,t450,t454,t457,t458,t460,t461,t462,t463,t464,t467,t468,t47,t470,t471,t473,t476,t479,t480,t481,t482,t483,t484,t485,t488,t49,t490,t491,t492,t493,t494,t495,t496,t497,t498,t499,t5,t50,t500,t501,t502,t503,t504,t505,t506,t507,t508,t509,t51,t510,t511,t512,t513,t514,t515,t516,t517,t518,t519,t52,t520,t521,t522,t523,t524,t525,t526,t527,t528,t529,t53,t530,t532,t533,t535,t536,t537,t538,t539,t54,t540,t541,t542,t543,t544,t545,t546,t547,t548,t549,t55,t550,t552,t553,t554,t555,t556,t557,t558,t559,t56,t560,t561,t565,t567,t568,t569,t57,t570,t571,t572,t573,t576,t578,t579,t58,t580,t585,t586,t588,t589,t59,t590,t591,t593,t595,t596,t598,t599,t6,t60,t600,t601,t608,t609,t61,t610,t612,t613,t614,t615,t619,t62,t620,t621,t625,t626,t627,t63,t630,t631,t634,t636,t637,t638,t639,t64,t642,t643,t645,t646,t647,t648,t65,t650,t651,t652,t653,t655,t656,t657,t66,t661,t662,t666,t668,t669,t67,t671,t672,t674,t675,t677,t678,t679,t68,t682,t685,t688,t689,t69,t690,t692,t693,t695,t697,t699,t7,t70,t701,t702,t706,t71,t711,t713,t718,t719,t72,t721,t723,t725,t727,t73,t732,t733,t734,t735,t736,t737,t738,t74,t740,t741,t742,t743,t747,t748,t749,t75,t752,t753,t754,t755,t756,t759,t76,t760,t761,t762,t763,t766,t767,t768,t77,t774,t78,t781,t783,t784,t785,t789,t79,t791,t792,t793,t794,t795,t796,t797,t798,t799,t8,t80,t800,t801,t802,t803,t804,t805,t806,t807,t808,t809,t81,t810,t811,t812,t813,t814,t815,t816,t817,t818,t819,t820,t821,t822,t823,t824,t825,t826,t827,t828,t829,t830,t831,t832,t833,t834,t835,t836,t837,t838,t839,t840,t841,t842,t843,t844,t845,t846,t847,t848,t849,t85,t850,t851,t852,t853,t854,t855,t856,t857,t858,t859,t86,t860,t861,t862,t863,t864,t865,t866,t867,t868,t869,t87,t870,t871,t872,t873,t874,t875,t876,t877,t878,t879,t88,t880,t881,t882,t883,t884,t885,t886,t887,t89,t891,t892,t893,t895,t896,t897,t899,t9,t90,t900,t902,t903,t904,t905,t906,t908,t909,t910,t912,t913,t917,t918,t919,t92,t920,t922,t927,t928,t929,t93,t930,t931,t932,t933,t934,t939,t94,t947,t948,t949,t950,t951,t952,t953,t954,t956,t957,t958,t959,t96,t961,t965,t966,t967,t968,t969,t97,t970,t971,t973,t974,t975,t976,t978,t979,t980,t983,t985,t987,t989,t99,t990,t994,t995,t996,t997] = ct{:};
t1465 = -t1258;
t1466 = -t1259;
t1470 = t3*t4*t967;
t1471 = -t1266;
t1472 = -t1269;
t1473 = -t1272;
t1476 = t36*t900;
t1477 = -t1278;
t1478 = t7*t12*t13*t540;
t1480 = t36*t639*2.0;
t1512 = t36*t747*2.0;
t1522 = t3*t10*t11*t552;
t1523 = t4*t9*t11*t552;
t1528 = t35*t949;
t1529 = t35*t950;
t1530 = t35*t951;
t1531 = t35*t952;
t1532 = t35*t953;
t1533 = t35*t954;
t1541 = t35*t957;
t1546 = -t1331;
t1547 = -t1332;
t1560 = t5*t1257;
t1561 = t5*t1258;
t1562 = t5*t1259;
t1571 = t9*t10*t947;
t1576 = -t1484;
t1577 = -t1487;
t1578 = -t1392;
t1579 = -t1393;
t1581 = -t1490;
t1582 = -t1491;
t1585 = t42*t47*t510;
t1592 = -t1409;
t1602 = -t1538;
t1603 = -t1539;
t1612 = t3*t5*t10*t11*t491;
t1613 = t4*t5*t9*t11*t491;
t1616 = -t1549;
t1619 = -t1554;
t1620 = -t1555;
t1624 = t3*t4*t36*t561;
t1625 = Lx3*t1507;
t1626 = t132+t554;
t1627 = t35*t36*t540;
t1631 = t11*t12*t36*t572;
t1635 = t3*t6*t10*t12*t553;
t1636 = t4*t6*t9*t12*t553;
t1640 = Lx3*t1540;
t1670 = t34*t36*t561;
t1673 = -t1553;
t1675 = -t1564;
t1676 = -t1565;
t1678 = -t1569;
t1679 = -t1570;
t1680 = t34*t1258*2.0;
t1681 = t34*t1259*2.0;
t1682 = t34*t1264*2.0;
t1683 = t34*t1265*2.0;
t1684 = -t1652;
t1686 = t5*t1507;
t1687 = -t1663;
t1688 = -t1664;
t1689 = -t1665;
t1690 = -t1666;
t1691 = -t1667;
t1692 = -t1668;
t1693 = t11*t1507;
t1694 = t5*t1540;
t1695 = t11*t1540;
t1696 = t11*t35*t49*t330;
t1701 = -t1618;
t1702 = -t1630;
t1703 = -t1632;
t1704 = -t1633;
t1708 = -t1637;
t1711 = t11*t35*t49*t552;
t1742 = t90+t146+t150+t240+t481+t485+t515+t517+t519+t547+t589+t967;
t1743 = t103+t266+t269+t450+t458+t480+t484+t506+t514+t516+t529+t814+t822+t828+t859;
t1386 = -t1069;
t1444 = t35*t880;
t1447 = t3*t4*t796;
t1448 = t3*t4*t799;
t1454 = t3*t4*t821;
t1455 = t3*t4*t827;
t1467 = -t1378;
t1468 = -t1261;
t1469 = -t1262;
t1479 = t11*t12*t966;
t1548 = -t1333;
t1580 = -t1395;
t1583 = -t1399;
t1584 = -t1400;
t1598 = -t1512;
t1634 = t36*t1260;
t1642 = t36*t1280;
t1643 = t11*t49*t906;
t1644 = t3*t10*t11*t906;
t1645 = t4*t9*t11*t906;
t1646 = -t1528;
t1647 = -t1529;
t1648 = -t1530;
t1649 = -t1531;
t1650 = -t1532;
t1651 = -t1533;
t1674 = t3*t4*t1297;
t1677 = t5*t1478;
t1697 = t35*t1431;
t1698 = t35*t1432;
t1706 = -t1682;
t1707 = -t1683;
t1709 = t11*t12*t36*t965;
t1710 = t1626^2;
t1712 = t35*t1522;
t1713 = t35*t1523;
t1725 = t69+t1693;
t1726 = t68+t1694;
t1732 = -Lx4*(t70-t1686);
t1734 = -t12*(t70-t1686);
t1736 = t6*(t70-t1686);
t1744 = t462+t810+t852+t856+t1081+t1114+t1743;
t1745 = t43+t44+t80+t92+t96+t97+t122+t125+t127+t129+t130+t131+t157+t179+t180+t212+t215+t221+t223+t330+t340+t407+t504+t509+t532+t552+t812+t819+t834+t860+t866+t876+t878+t906+t948+t1203+t1290;
t1749 = t168+t337+t338+t463+t521+t572+t573+t613+t661+t666+t736+t793+t795+t802+t806+t839+t840+t855+t965+t966+t1036+t1060+t1076+t1079+t1111+t1112+t1119+t1120+t1121+t1128+t1129+t1130+t1147+t1148+t1152+t1155+t1156+t1160+t1216+t1217+t1219+t1220+t1288+t1289+t1295+t1296+t1344+t1349+t1351+t1354+t1356+t1366+t1368+t1383+t1384+t1453;
t1750 = t233+t234+t237+t238+t368+t375+t382+t386+t457+t467+t579+t580+t585+t586+t590+t591+t595+t596+t598+t599+t600+t601+t637+t638+t643+t648+t653+t679+t697+t699+t718+t719+t721+t732+t738+t752+t753+t759+t760+t766+t767+t774+t781+t784+t789+t798+t817+t845+t869+t891+t892+t1002+t1003+t1013+t1015+t1017+t1020+t1024+t1027+t1032+t1044+t1046+t1049+t1051+t1061+t1066+t1068+t1084+t1085+t1091+t1094+t1097+t1106+t1113+t1142+t1144+t1146+t1162+t1210+t1211+t1257+t1281+t1311+t1328+t1329+t1341+t1342+t1345+t1365+t1367+t1369+t1370+t1387+t1443+t1470+t1478+t1481+t1482+t1546+t1547+t1561+t1562+t1675+t1676;
t1705 = -t1634;
t1723 = t35*t1644;
t1724 = t35*t1645;
t1727 = Lx4*t1726;
t1730 = t12*t1726;
t1731 = t6*t1726;
t1739 = t1604+t1734;
t1740 = t1605+t1736;
t1746 = t178+t213+t217+t219+t339+t377+t384+t388+t740+t809+t846+t1115+t1745;
t1747 = t99+t145+t151+t152+t209+t226+t230+t242+t243+t253+t412+t449+t483+t510+t511+t512+t513+t518+t520+t530+t533+t588+t593+t619+t796+t799+t821+t827+t833+t867+t868+t893+t895+t896+t939+t968+t969+t970+t980+t1205+t1206+t1212+t1297+t1330+t1371+t1548;
t1751 = Ixx4+Iyy3+Izz5+Izz6+t50+t52+t53+t54+t55+t56+t57+t58+t59+t60+t61+t63+t64+t75+t76+t77+t78+t79+t93+t94+t105+t106+t108+t109+t110+t118+t119+t120+t121+t147+t148+t163+t164+t165+t166+t167+t171+t173+t175+t177+t214+t218+t220+t276+t277+t278+t279+t280+t281+t282+t290+t291+t292+t293+t294+t295+t299+t302+t303+t304+t336+t345+t346+t347+t348+t376+t383+t387+t464+t488+t490+t492+t493+t495+t500+t505+t527+t528+t546+t548+t549+t550+t556+t557+t558+t559+t560+t561+t565+t576+t578+t615+t804+t811+t813+t818+t823+t829+t850+t857+t858+t865+t879+t880+t881+t882+t910+t956+t957+t959+t961+t971+t983+t985+t1080+t1101+t1124+t1133+t1153+t1161+t1166+t1196+t1202+t1204+t1300+t1301+t1302+t1303+t1304+t1315+t1319+t1379+t1426+t1437+t1438+t1444+t1467+t1541+t1572+t1670;
t1752 = t187+t188+t349+t351+t352+t400+t401+t420+t421+t422+t423+t431+t432+t454+t470+t476+t479+t620+t621+t668+t669+t688+t689+t690+t733+t734+t735+t797+t820+t824+t830+t883+t884+t885+t886+t887+t912+t913+t919+t920+t927+t928+t933+t934+t994+t995+t996+t997+t1004+t1005+t1065+t1073+t1074+t1075+t1095+t1167+t1168+t1171+t1184+t1187+t1188+t1189+t1221+t1223+t1224+t1236+t1237+t1238+t1239+t1285+t1291+t1292+t1343+t1360+t1361+t1388+t1394+t1402+t1403+t1404+t1405+t1406+t1407+t1408+t1411+t1412+t1421+t1428+t1435+t1436+t1439+t1440+t1441+t1442+t1445+t1446+t1450+t1451+t1456+t1460+t1461+t1462+t1506+t1508+t1535+t1536+t1537+t1543+t1551+t1552+t1573+t1574+t1578+t1579+t1585+t1592+t1593+t1594+t1595+t1596+t1597+t1600+t1601+t1607+t1616+t1617+t1623+t1628+t1629+t1638+t1639+t1643+t1653+t1654+t1662+t1673+t1684+t1687+t1688+t1696+t1699+t1700+t1701+t1702+t1708+t1711+t1716+t1720;
et1 = t71+t72+t73+t153+t154+t155+t170+t172+t174+t176+t298+t300+t305+t306+t307+t308+t309+t310+t311+t312+t313+t314+t319+t322+t323+t324+t326+t327+t331+t332+t333+t334+t335+t374+t379+t380+t381+t385+t392+t393+t460+t461+t494+t499+t526+t535+t536+t537+t538+t539+t540+t541+t542+t543+t544+t545+t555+t567+t568+t569+t608+t609+t610+t612+t614+t625+t626+t627+t642+t645+t646+t647+t650+t651+t652+t655+t656+t671+t672+t677+t678+t711+t713+t725+t727+t737+t742+t743+t791+t800+t801+t803+t825+t826+t841+t842+t843+t844+t848+t849+t861+t862+t871+t873+t875+t897+t899+t902+t903+t904+t905+t908+t909+t922+t987+t989+t990+t1035+t1038+t1041+t1057+t1058+t1070+t1077+t1078+t1082+t1089+t1090+t1092+t1093+t1102+t1103+t1104+t1105+t1107+t1108+t1109+t1110+t1117+t1125+t1126+t1134+t1138+t1139+t1140+t1141+t1143+t1145+t1154+t1194+t1199+t1231+t1232+t1233+t1234+t1235+t1267+t1268+t1270+t1271+t1273+t1274+t1275+t1276+t1317+t1318+t1334+t1335+t1336+t1337+t1338+t1339+t1346+t1347+t1348+t1350+t1352+t1353+t1355+t1357+t1358+t1372+t1373+t1374+t1375+t1376+t1377+t1380+t1381+t1386+t1391+t1396+t1397+t1452+t1458+t1463+t1464+t1468+t1469+t1476;
et2 = t1485+t1486+t1488+t1489+t1510+t1511+t1513+t1566+t1567+t1575+t1583+t1584+t1586+t1587+t1588+t1589+t1624+t1627+t1635+t1636+t1656+t1657+t1678+t1679+t1703+t1704;
t1753 = et1+et2;
t1735 = -t1731;
t1737 = t1606+t1730;
t1748 = t496+t501+t522+t523+t524+t525+t741+t805+t847+t851+t870+t872+t874+t1116+t1747;
et3 = t86+t87+t89+t144+t189+t190+t192+t198+t205+t206+t244+t246+t248+t250+t257+t351+t352+t354+t355+t358+t372+t373+t394+t404+t405+t408+t409+t410+t411+t422+t423+t425+t426+t428+t429+t431+t432+t435+t439+t454+t468+t470+t471+t473+t476+t482+t497+t498+t502+t503+t507+t508+t630+t631+t636+t657+t662+t674+t675+t682+t685+t692+t693+t695+t701+t702+t706+t723+t747+t748+t749+t754+t755+t756+t761+t762+t763+t768+t783+t785+t792+t794+t797+t807+t808+t815+t816+t820+t824+t831+t832+t835+t836+t837+t838+t853+t854+t863+t864+t877+t912+t913+t917+t918+t927+t928+t929+t930+t931+t932+t933+t934+t949+t950+t951+t952+t953+t954+t973+t974+t975+t976+t978+t979+t1001+t1008+t1009+t1011+t1022+t1029+t1048+t1053+t1056+t1067+t1072+t1083+t1086+t1087+t1088+t1096+t1098+t1099+t1100+t1118+t1122+t1123+t1127+t1131+t1132+t1136+t1137+t1149+t1150+t1151+t1157+t1158+t1159+t1163+t1164+t1165+t1178+t1179+t1180+t1181+t1182+t1183+t1226+t1227+t1246+t1247+t1248+t1249+t1250+t1251+t1254+t1260+t1264+t1265+t1277+t1282+t1283+t1284+t1286+t1287+t1291+t1292+t1293+t1294+t1305+t1306+t1307+t1308+t1320+t1321+t1323+t1324+t1327+t1340+t1359+t1362;
et4 = t1363+t1364+t1382+t1385+t1398+t1417+t1422+t1423+t1424+t1425+t1427+t1429+t1430+t1431+t1432+t1433+t1434+t1447+t1448+t1454+t1455+t1465+t1466+t1471+t1472+t1473+t1477+t1479+t1480+t1492+t1493+t1494+t1496+t1498+t1499+t1501+t1503+t1514+t1515+t1516+t1517+t1518+t1519+t1520+t1521+t1522+t1523+t1524+t1525+t1544+t1545+t1558+t1559+t1560+t1571+t1576+t1577+t1580+t1581+t1582+t1590+t1591+t1598+t1599+t1602+t1603+t1612+t1613+t1619+t1620+t1621+t1622+t1631+t1642+t1644+t1645+t1646+t1647+t1648+t1649+t1650+t1651+t1658+t1659+t1660+t1661+t1669+t1671+t1672+t1674+t1677+t1680+t1681+t1685+t1689+t1690+t1691+t1692+t1697+t1698+t1705+t1706+t1707+t1709+t1712+t1713+t1721+t1722+t1723+t1724;
t1754 = et3+et4;
t1738 = t1608+t1735;
et5 = Izz1+Ixx3*t117+Izz3*t116+Izz4*t116+Izz5*t1710+Izz6*t1710+m2*(t74-Lycm2*t8+Lxcm2*t2*t3+Lzcm2*t2*t9)^2+m2*(t85+Lycm2*t2+Lxcm2*t3*t8+Lzcm2*t8*t9)^2+m5*(t74+t1625+t1732-Lxcm5*t1740-Lycm5*t1725+Lzcm5*t1739)^2+t104*t117+m6*(t74+t1625+t1732+Lz6*t1739+Lzcm6*t1739-Lxcm6*(t13*t1725+t7*t1740)-Lycm6*(t7*t1725-t13*t1740))^2+Ixx6*(t7*t1474-t11*t13*t49)^2+Iyy6*(t13*t1474+t7*t11*t49)^2+m4*(t74+t1625+t1732-Lycm4*t1725+Lzcm4*t1298-Lxcm4*(t70-t1686))^2+m4*(t85+t1640+t1727+Lxcm4*t1726+Lzcm4*t1299+Lycm4*(t67-t1695))^2;
et6 = m5*(t85+t1640+t1727-Lxcm5*t1738+Lzcm5*t1737+Lycm5*(t67-t1695))^2+Ixx2*t9^2+Ixx5*t1474^2+Izz2*t3^2+m6*(t85+t1640+t1727+Lz6*t1737+Lzcm6*t1737-Lxcm6*(t7*t1738-t13*(t67-t1695))+Lycm6*(t13*t1738+t7*(t67-t1695)))^2+m1*(Lxcm1*t8+Lycm1*t2)^2+m1*(Lxcm1*t2-Lycm1*t8)^2+m3*(t74+t1625+Lxcm3*t1507-Lycm3*t8+Lzcm3*t1298)^2+m3*(t85+t1640+Lxcm3*t1540+Lycm3*t2+Lzcm3*t1299)^2+Iyy4*t40*t117+Iyy5*t40*t117;
et7 = Ixx4+Iyy2+Iyy3+Izz5+Izz6+t50+t52+t53+t54+t55+t56+t57+t58+t59+t60+t61+t63+t64+t75*2.0+t76*2.0+t77*2.0+t78*2.0+t79*2.0+t93*2.0+t94*2.0+t105+t106+t108+t109+t110+t118+t119+t120+t121+t147+t148+t163+t164+t165+t166+t167+t171*2.0+t173*2.0+t175*2.0+t177*2.0-t193*2.0-t199*2.0+t214*2.0+t218*2.0+t220*2.0-t252*2.0+t276+t277+t278+t279+t280+t281+t282+t290+t291+t292+t293+t294+t295+t299+t302+t303+t304+t336*2.0+t345+t346+t347+t348-t359*2.0+t376*2.0+t383*2.0+t387*2.0-t440*2.0-t447*2.0+t464*2.0+t488+t490+t492+t493+t505+t528+t546+t548+t549+t550+t556+t557+t558+t559+t560+t561+t565+t576+t578+t615*2.0-t634*2.0+t811+t813+t818+t823+t829+t858+t865+t879+t880+t881+t882+t910+t956+t957+t959+t961+t971+t983+t985+t1101+t1124+t1133+t1153+t1161+t1166+t1196+t1202+t1204+t1300+t1301+t1302+t1303+t1304+t1315+t1319+t1379+t1426+t1437;
et8 = t1438+t1444+t1467+t1541+t1572+t1670+m2*t15+m3*t15+m4*t15+m5*t15+m6*t15+Lxcm2^2*m2+Lzcm2^2*m2+Lx2*Lxcm2*m2*2.0;
mt1 = [et5+et6,t1754,t1752,t1753,t1750,t1749,t1754,et7+et8,t1751,t1748,t1746,t1744,t1752,t1751,Ixx4+Iyy3+Izz5+Izz6+t50+t52+t53+t54+t55+t56+t57+t58+t59+t60+t61+t63+t64+t105+t106+t108+t109+t110+t118+t119+t120+t121+t147+t148+t163+t164+t165+t166+t167+t276+t277+t278+t279+t280+t281+t282+t290+t291+t292+t293+t294+t295+t299+t302+t303+t304+t345+t346+t347+t348+t488+t490+t492+t493+t505+t528+t546+t548+t549+t550+t556+t557+t558+t559+t560+t561+t565+t576+t578+t811+t813+t818+t823+t829+t858+t865+t879+t880+t881+t882+t910+t956+t957+t959+t961+t971+t983+t985+t1101+t1124+t1133+t1153+t1161+t1166+t1196+t1202+t1204+t1300+t1301+t1302+t1303+t1304+t1315+t1319+t1379+t1426+t1437+t1438+t1444+t1467+t1541+t1572+t1670,t1747,t1745,t1743,t1753,t1748,t1747];
mt2 = [Ixx5+Iyy6+Izz4+t51+t58+t59+t60+t62+t65+t66-t105+t107-t110-t111+t113+t115+t161+t162+t283-t285+t288+t289-t291-t293-t295-t488+t491+t570+t571-t576-t578+t958-t983+m4*t17+m5*t17+m4*t19+m6*t17+t6*t81*2.0-t6*t88*2.0+t36*t561+Lx4*Lxcm4*m4*2.0+Lx4*Lxcm5*m5*t6*2.0+Lx4*Lz6*m6*t12*2.0+Lx4*Lzcm5*m5*t12*2.0+Lx4*Lzcm6*m6*t12*2.0-Lz6*Lzcm6*m6*t35*2.0,t1742,t1741,t1750,t1746,t1745,t1742,Ixx6+Iyy5+t51+t57+t61+t62+t65+t66-t107+t111-t161+t285-t289,t1449,t1749,t1744,t1743,t1741,t1449,Izz6+t58+t61];
out1 = reshape([mt1,mt2],6,6);
end
